simulink model "pokus07_video"  (R2023a)
settings: Solver=VariableStepAuto  StartTime=0.0  StopTime=10.0  RelTol=1e-3
undefined symbols (not defined in the file): c
libraries: Miscellaneous x840, Memory_Blocks_Lib x251, Decoders_Lib x10, simulink_extras x10, Counters_Lib x4, Bit_Multiplexers_Lib x1, Byte_Multiplexers_Lib x1
(part 3 of 5)

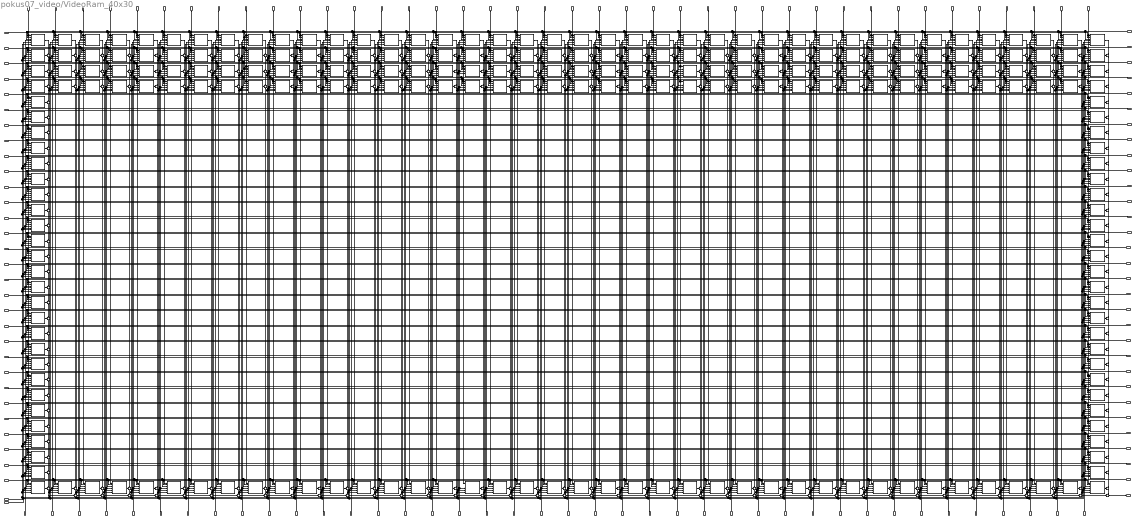
== system pokus07_video/VideoRam_40x30 ==
  RR29 : Inport
  RR28 : Inport  Port=2
  RR27 : Inport  Port=3
  RR26 : Inport  Port=4
  RR25 : Inport  Port=5
  RR24 : Inport  Port=6
  RR23 : Inport  Port=7
  RR22 : Inport  Port=8
  RR21 : Inport  Port=9
  RR20 : Inport  Port=10
  RR19 : Inport  Port=11
  RR18 : Inport  Port=12
  RR17 : Inport  Port=13
  RR16 : Inport  Port=14
  RR15 : Inport  Port=15
  RR14 : Inport  Port=16
  RR13 : Inport  Port=17
  RR12 : Inport  Port=18
  RR11 : Inport  Port=19
  RR10 : Inport  Port=20
  RR09 : Inport  Port=21
  RR08 : Inport  Port=22
  RR07 : Inport  Port=23
  RR06 : Inport  Port=24
  RR05 : Inport  Port=25
  RR04 : Inport  Port=26
  RR03 : Inport  Port=27
  RR02 : Inport  Port=28
  RR01 : Inport  Port=29
  RR00 : Inport  Port=30
  OrdNumIn(2B) : Inport  Port=31
  CLK : Inport  Port=32
  RC39 : Inport  Port=33
  RC38 : Inport  Port=34
  RC37 : Inport  Port=35
  RC36 : Inport  Port=36
  RC35 : Inport  Port=37
  RC34 : Inport  Port=38
  RC33 : Inport  Port=39
  RC32 : Inport  Port=40
  RC31 : Inport  Port=41
  RC30 : Inport  Port=42
  RC29 : Inport  Port=43
  RC28 : Inport  Port=44
  RC27 : Inport  Port=45
  RC26 : Inport  Port=46
  RC25 : Inport  Port=47
  RC24 : Inport  Port=48
  RC23 : Inport  Port=49
  RC22 : Inport  Port=50
  RC21 : Inport  Port=51
  RC20 : Inport  Port=52
  RC19 : Inport  Port=53
  RC18 : Inport  Port=54
  RC17 : Inport  Port=55
  RC16 : Inport  Port=56
  RC15 : Inport  Port=57
  RC14 : Inport  Port=58
  RC13 : Inport  Port=59
  RC12 : Inport  Port=60
  RC11 : Inport  Port=61
  RC10 : Inport  Port=62
  RC09 : Inport  Port=63
  RC08 : Inport  Port=64
  RC07 : Inport  Port=65
  RC06 : Inport  Port=66
  RC05 : Inport  Port=67
  RC04 : Inport  Port=68
  RC03 : Inport  Port=69
  RC02 : Inport  Port=70
  RC01 : Inport  Port=71
  RC00 : Inport  Port=72
  WC39 : Inport  Port=73
  WC38 : Inport  Port=74
  WC37 : Inport  Port=75
  WC36 : Inport  Port=76
  WC35 : Inport  Port=77
  WC34 : Inport  Port=78
  WC33 : Inport  Port=79
  WC32 : Inport  Port=80
  WC31 : Inport  Port=81
  WC30 : Inport  Port=82
  WC29 : Inport  Port=83
  WC28 : Inport  Port=84
  WC27 : Inport  Port=85
  WC26 : Inport  Port=86
  WC25 : Inport  Port=87
  WC24 : Inport  Port=88
  WC23 : Inport  Port=89
  WC22 : Inport  Port=90
  WC21 : Inport  Port=91
  WC20 : Inport  Port=92
  WC19 : Inport  Port=93
  WC18 : Inport  Port=94
  WC17 : Inport  Port=95
  WC16 : Inport  Port=96
  WC15 : Inport  Port=97
  WC14 : Inport  Port=98
  WC13 : Inport  Port=99
  WC12 : Inport  Port=100
  WC11 : Inport  Port=101
  WC10 : Inport  Port=102
  WC09 : Inport  Port=103
  WC08 : Inport  Port=104
  WC07 : Inport  Port=105
  WC06 : Inport  Port=106
  WC05 : Inport  Port=107
  WC04 : Inport  Port=108
  WC03 : Inport  Port=109
  WC02 : Inport  Port=110
  WC01 : Inport  Port=111
  WC00 : Inport  Port=112
  WR29 : Inport  Port=113
  WR28 : Inport  Port=114
  WR27 : Inport  Port=115
  WR26 : Inport  Port=116
  WR25 : Inport  Port=117
  WR24 : Inport  Port=118
  WR23 : Inport  Port=119
  WR22 : Inport  Port=120
  WR21 : Inport  Port=121
  WR20 : Inport  Port=122
  WR19 : Inport  Port=123
  WR18 : Inport  Port=124
  WR17 : Inport  Port=125
  WR16 : Inport  Port=126
  WR15 : Inport  Port=127
  WR14 : Inport  Port=128
  WR13 : Inport  Port=129
  WR12 : Inport  Port=130
  WR11 : Inport  Port=131
  WR10 : Inport  Port=132
  WR09 : Inport  Port=133
  WR08 : Inport  Port=134
  WR07 : Inport  Port=135
  WR06 : Inport  Port=136
  WR05 : Inport  Port=137
  WR04 : Inport  Port=138
  WR03 : Inport  Port=139
  WR02 : Inport  Port=140
  WR01 : Inport  Port=141
  WR00 : Inport  Port=142
  Byte_TwoBusAccess{,1..249} (250 alike) : Memory_Blocks_Lib/Byte_TwoBusAccess  SystemSampleTime=-1  VariantActivationTime=update diagram  Latency=0  AutoFrameSizeCalculation=off
  Merge2_Simulated{1..15,17..64,66..67,74..75,88..89,92..93,100,102,105..107,112..114,116..117,123..124,126..127,129..131,133..137,140..146,151,154..155,158..161,163..164,167..174,179,184,189,191..193,195..201,203..205,207..209,211..213,215,217..219,222..225,227..233,235..237,239..241,243..245,247,249..251,254..257,259..265,267..269,271..273,275..277,279,281..283,286..289,291..297,299..301,303..305,307..309,311..348} (249 alike) : Miscellaneous/Merge2_Simulated  SystemSampleTime=-1  VariantActivationTime=update diagram  Latency=0  AutoFrameSizeCalculation=off
      settings: PortSchema="{\"entries\":[{\"content\":{\"sides\":[{\"content\":{\"connectorIds\":[\"In1\"]},\"type\":\"ConnectorPlacement.EquallySpacedRectSide\",\"uuid\":\"74758995-5ec8-49f8-a534-c3a678c5c312\"},{\"content\":{\"side\":\"RIGHT\"},\"type\":\"ConnectorPlacement.EquallySpacedRectSide\",\"uuid\":\"c467dbeb-9f00-48b9-a78d-a08162163a10\"},{\"content\":{\"connectorIds\":[\"Out1\"],\"side\":\"TOP\"},\"type\":\"ConnectorPlacement.EquallySpacedRectSide\",\"uuid\":\"39dea3b5-6733-4ade-ab22-e62d310be187\"},{\"content\":{\"connectorIds\":[\"In2\"],\"side\":\"BOTTOM\"},\"type\":\"ConnectorPlacement.EquallySpacedRectSide\",\"uuid\":\"73149fc1-24d9-4bdc-92e2-12fb1d742836\"}]},\"type\":\"ConnectorPlacement.EquallySpacedConnector\",\"uuid\":\"fd2226dc-a4d3-43ad-9cda-54babd09ac78\"}],\"packageUris\":[\"http://schema.mathworks.com/mf0/Connector/R2020b\"],\"version\":\"1.0\"}"
  OrdNumOut(1B) : Outport
  wires:
  Byte_TwoBusAccess52/1 -> Merge2_Simulated1/1
  Byte_TwoBusAccess132/1 -> Merge2_Simulated3/1
  Byte_TwoBusAccess92/1 -> Merge2_Simulated2/1
  Merge2_Simulated2/1 -> Merge2_Simulated3/2
  Merge2_Simulated1/1 -> Merge2_Simulated2/2
  Byte_TwoBusAccess2/1 -> Merge2_Simulated1/2
  Byte_TwoBusAccess121/1 -> Merge2_Simulated7/1
  Merge2_Simulated5/1 -> Merge2_Simulated6/2
  Byte_TwoBusAccess1/1 -> Merge2_Simulated5/2
  Byte_TwoBusAccess81/1 -> Merge2_Simulated6/1
  Byte_TwoBusAccess41/1 -> Merge2_Simulated5/1
  Merge2_Simulated6/1 -> Merge2_Simulated7/2
  Byte_TwoBusAccess120/1 -> Merge2_Simulated11/1
  Merge2_Simulated9/1 -> Merge2_Simulated10/2
  Byte_TwoBusAccess/1 -> Merge2_Simulated9/2
  Byte_TwoBusAccess80/1 -> Merge2_Simulated10/1
  Byte_TwoBusAccess40/1 -> Merge2_Simulated9/1
  Merge2_Simulated10/1 -> Merge2_Simulated11/2
  Byte_TwoBusAccess143/1 -> Merge2_Simulated15/1
  Merge2_Simulated13/1 -> Merge2_Simulated14/2
  Byte_TwoBusAccess3/1 -> Merge2_Simulated13/2
  Byte_TwoBusAccess103/1 -> Merge2_Simulated14/1
  Byte_TwoBusAccess63/1 -> Merge2_Simulated13/1
  Merge2_Simulated14/1 -> Merge2_Simulated15/2
  Merge2_Simulated18/1 -> Merge2_Simulated19/2
  Merge2_Simulated30/1 -> Merge2_Simulated31/2
  Merge2_Simulated31/1 -> Merge2_Simulated18/2
  Byte_TwoBusAccess228/1 -> Merge2_Simulated19/1
  Byte_TwoBusAccess225/1 -> Merge2_Simulated30/1
  Byte_TwoBusAccess227/1 -> Merge2_Simulated18/1
  Byte_TwoBusAccess226/1 -> Merge2_Simulated31/1
  RC01/1 -> Byte_TwoBusAccess1/1, Byte_TwoBusAccess41/1, Byte_TwoBusAccess81/1, Byte_TwoBusAccess161/1, Byte_TwoBusAccess121/1
  Merge2_Simulated11/1 -> Merge2_Simulated30/2
  Merge2_Simulated34/1 -> Merge2_Simulated35/2
  Merge2_Simulated62/1 -> Merge2_Simulated63/2
  Merge2_Simulated63/1 -> Merge2_Simulated34/2
  Byte_TwoBusAccess235/1 -> Merge2_Simulated42/1
  Byte_TwoBusAccess236/1 -> Merge2_Simulated43/1
  Byte_TwoBusAccess234/1 -> Merge2_Simulated57/1
  Merge2_Simulated56/1 -> Merge2_Simulated57/2
  Byte_TwoBusAccess229/1 -> Merge2_Simulated62/1
  Byte_TwoBusAccess231/1 -> Merge2_Simulated34/1
  Byte_TwoBusAccess230/1 -> Merge2_Simulated63/1
  Byte_TwoBusAccess232/1 -> Merge2_Simulated35/1
  Merge2_Simulated35/1 -> Merge2_Simulated56/2
  Merge2_Simulated57/1 -> Merge2_Simulated42/2
  Merge2_Simulated42/1 -> Merge2_Simulated43/2
  Byte_TwoBusAccess233/1 -> Merge2_Simulated56/1
  Merge2_Simulated19/1 -> Merge2_Simulated62/2
  Merge2_Simulated66/1 -> Merge2_Simulated67/2
  Merge2_Simulated126/1 -> Merge2_Simulated127/2
  Merge2_Simulated127/1 -> Merge2_Simulated66/2
  Merge2_Simulated75/1 -> Merge2_Simulated123/2
  Byte_TwoBusAccess249/1 -> Merge2_Simulated116/1
  Merge2_Simulated93/1 -> Merge2_Simulated116/2
  Byte_TwoBusAccess160/1 -> Merge2_Simulated117/1
  Byte_TwoBusAccess183/1 -> Merge2_Simulated105/1
  Merge2_Simulated124/1 -> Merge2_Simulated92/2
  Merge2_Simulated123/1 -> Merge2_Simulated124/2
  Merge2_Simulated92/1 -> Merge2_Simulated93/2
  Byte_TwoBusAccess245/1 -> Merge2_Simulated123/1
  Merge2_Simulated15/1 -> Merge2_Simulated105/2
  Merge2_Simulated116/1 -> Merge2_Simulated117/2
  WC01/1 -> Byte_TwoBusAccess161/4, Byte_TwoBusAccess121/4, Byte_TwoBusAccess81/4, Byte_TwoBusAccess41/4, Byte_TwoBusAccess1/4
  WC00/1 -> Byte_TwoBusAccess160/4, Byte_TwoBusAccess249/4, Byte_TwoBusAccess248/4, Byte_TwoBusAccess247/4, Byte_TwoBusAccess246/4, Byte_TwoBusAccess245/4, Byte_TwoBusAccess244/4, Byte_TwoBusAccess243/4, Byte_TwoBusAccess242/4, Byte_TwoBusAccess241/4, Byte_TwoBusAccess240/4, Byte_TwoBusAccess239/4, Byte_TwoBusAccess238/4, Byte_TwoBusAccess237/4, Byte_TwoBusAccess236/4, Byte_TwoBusAccess235/4, Byte_TwoBusAccess234/4, Byte_TwoBusAccess233/4, Byte_TwoBusAccess232/4, Byte_TwoBusAccess231/4, Byte_TwoBusAccess230/4, Byte_TwoBusAccess229/4, Byte_TwoBusAccess228/4, Byte_TwoBusAccess227/4, Byte_TwoBusAccess226/4, Byte_TwoBusAccess225/4, Byte_TwoBusAccess120/4, Byte_TwoBusAccess80/4, Byte_TwoBusAccess40/4, Byte_TwoBusAccess/4
  Merge2_Simulated7/1 -> Merge2_Simulated112/2
  Byte_TwoBusAccess172/1 -> Merge2_Simulated100/1
  Merge2_Simulated3/1 -> Merge2_Simulated100/2
  Byte_TwoBusAccess243/1 -> Merge2_Simulated74/1
  Byte_TwoBusAccess244/1 -> Merge2_Simulated75/1
  Byte_TwoBusAccess242/1 -> Merge2_Simulated89/1
  Merge2_Simulated88/1 -> Merge2_Simulated89/2
  Byte_TwoBusAccess237/1 -> Merge2_Simulated126/1
  Byte_TwoBusAccess239/1 -> Merge2_Simulated66/1
  Byte_TwoBusAccess238/1 -> Merge2_Simulated127/1
  Byte_TwoBusAccess161/1 -> Merge2_Simulated112/1
  Byte_TwoBusAccess240/1 -> Merge2_Simulated67/1
  Merge2_Simulated67/1 -> Merge2_Simulated88/2
  Merge2_Simulated89/1 -> Merge2_Simulated74/2
  Byte_TwoBusAccess241/1 -> Merge2_Simulated88/1
  Merge2_Simulated74/1 -> Merge2_Simulated75/2
  Byte_TwoBusAccess246/1 -> Merge2_Simulated124/1
  RC02/1 -> Byte_TwoBusAccess2/1, Byte_TwoBusAccess52/1, Byte_TwoBusAccess92/1, Byte_TwoBusAccess172/1, Byte_TwoBusAccess132/1
  Byte_TwoBusAccess247/1 -> Merge2_Simulated92/1
  RC00/1 -> Byte_TwoBusAccess/1, Byte_TwoBusAccess40/1, Byte_TwoBusAccess80/1, Byte_TwoBusAccess120/1, Byte_TwoBusAccess225/1, Byte_TwoBusAccess226/1, Byte_TwoBusAccess227/1, Byte_TwoBusAccess228/1, Byte_TwoBusAccess229/1, Byte_TwoBusAccess230/1, Byte_TwoBusAccess231/1, Byte_TwoBusAccess232/1, Byte_TwoBusAccess233/1, Byte_TwoBusAccess234/1, Byte_TwoBusAccess235/1, Byte_TwoBusAccess236/1, Byte_TwoBusAccess237/1, Byte_TwoBusAccess238/1, Byte_TwoBusAccess239/1, Byte_TwoBusAccess240/1, Byte_TwoBusAccess241/1, Byte_TwoBusAccess242/1, Byte_TwoBusAccess243/1, Byte_TwoBusAccess244/1, Byte_TwoBusAccess245/1, Byte_TwoBusAccess246/1, Byte_TwoBusAccess247/1, Byte_TwoBusAccess248/1, Byte_TwoBusAccess249/1, Byte_TwoBusAccess160/1
  Byte_TwoBusAccess248/1 -> Merge2_Simulated93/1
  Merge2_Simulated43/1 -> Merge2_Simulated126/2
  Merge2_Simulated129/1 -> Merge2_Simulated140/2
  Byte_TwoBusAccess156/1 -> Merge2_Simulated151/1
  Merge2_Simulated133/1 -> Merge2_Simulated134/2
  Merge2_Simulated130/1 -> Merge2_Simulated131/2
  Byte_TwoBusAccess4/1 -> Merge2_Simulated191/2
  Merge2_Simulated191/1 -> Merge2_Simulated130/2
  Merge2_Simulated134/1 -> Merge2_Simulated135/2
  Merge2_Simulated184/1 -> Merge2_Simulated189/2
  Merge2_Simulated173/1 -> Merge2_Simulated184/2
  Byte_TwoBusAccess117/1 -> Merge2_Simulated134/1
  Byte_TwoBusAccess76/1 -> Merge2_Simulated129/1
  Byte_TwoBusAccess5/1 -> Merge2_Simulated173/2
  Byte_TwoBusAccess157/1 -> Merge2_Simulated135/1
  Byte_TwoBusAccess7/1 -> Merge2_Simulated133/2
  Byte_TwoBusAccess114/1 -> Merge2_Simulated130/1
  Byte_TwoBusAccess74/1 -> Merge2_Simulated191/1
  Byte_TwoBusAccess154/1 -> Merge2_Simulated131/1
  Byte_TwoBusAccess115/1 -> Merge2_Simulated184/1
  Byte_TwoBusAccess155/1 -> Merge2_Simulated189/1
  Byte_TwoBusAccess116/1 -> Merge2_Simulated140/1
  RC06/1 -> Byte_TwoBusAccess6/1, Byte_TwoBusAccess76/1, Byte_TwoBusAccess116/1, Byte_TwoBusAccess196/1, Byte_TwoBusAccess156/1
  Byte_TwoBusAccess75/1 -> Merge2_Simulated173/1
  Byte_TwoBusAccess6/1 -> Merge2_Simulated129/2
  RC04/1 -> Byte_TwoBusAccess4/1, Byte_TwoBusAccess74/1, Byte_TwoBusAccess114/1, Byte_TwoBusAccess194/1, Byte_TwoBusAccess154/1
  Byte_TwoBusAccess77/1 -> Merge2_Simulated133/1
  Merge2_Simulated140/1 -> Merge2_Simulated151/2
  WC13/1 -> Byte_TwoBusAccess165/4, Byte_TwoBusAccess125/4, Byte_TwoBusAccess85/4, Byte_TwoBusAccess45/4, Byte_TwoBusAccess13/4
  WC14/1 -> Byte_TwoBusAccess166/4, Byte_TwoBusAccess126/4, Byte_TwoBusAccess86/4, Byte_TwoBusAccess46/4, Byte_TwoBusAccess14/4
  WC15/1 -> Byte_TwoBusAccess167/4, Byte_TwoBusAccess127/4, Byte_TwoBusAccess87/4, Byte_TwoBusAccess47/4, Byte_TwoBusAccess15/4
  Byte_TwoBusAccess14/1 -> Merge2_Simulated113/2
  WC12/1 -> Byte_TwoBusAccess164/4, Byte_TwoBusAccess124/4, Byte_TwoBusAccess84/4, Byte_TwoBusAccess44/4, Byte_TwoBusAccess12/4
  Merge2_Simulated208/1 -> Merge2_Simulated209/2
  Byte_TwoBusAccess47/1 -> Merge2_Simulated195/1
  Byte_TwoBusAccess45/1 -> Merge2_Simulated203/1
  Byte_TwoBusAccess8/1 -> Merge2_Simulated215/2
  Merge2_Simulated207/1 -> Merge2_Simulated192/2
  Byte_TwoBusAccess12/1 -> Merge2_Simulated207/2
  Byte_TwoBusAccess119/1 -> Merge2_Simulated212/1
  Merge2_Simulated195/1 -> Merge2_Simulated196/2
  Byte_TwoBusAccess126/1 -> Merge2_Simulated201/1
  WC11/1 -> Byte_TwoBusAccess163/4, Byte_TwoBusAccess123/4, Byte_TwoBusAccess83/4, Byte_TwoBusAccess43/4, Byte_TwoBusAccess11/4
  Merge2_Simulated102/1 -> Merge2_Simulated208/2
  Byte_TwoBusAccess10/1 -> Merge2_Simulated102/2
  Byte_TwoBusAccess123/1 -> Merge2_Simulated200/1
  Merge2_Simulated212/1 -> Merge2_Simulated213/2
  Byte_TwoBusAccess122/1 -> Merge2_Simulated209/1
  Byte_TwoBusAccess127/1 -> Merge2_Simulated197/1
  Byte_TwoBusAccess46/1 -> Merge2_Simulated113/1
  Merge2_Simulated204/1 -> Merge2_Simulated205/2
  RC12/1 -> Byte_TwoBusAccess12/1, Byte_TwoBusAccess44/1, Byte_TwoBusAccess84/1, Byte_TwoBusAccess164/1, Byte_TwoBusAccess124/1
  Byte_TwoBusAccess43/1 -> Merge2_Simulated114/1
  Merge2_Simulated113/1 -> Merge2_Simulated199/2
  WC09/1 -> Byte_TwoBusAccess199/4, Byte_TwoBusAccess159/4, Byte_TwoBusAccess119/4, Byte_TwoBusAccess79/4, Byte_TwoBusAccess9/4
  Byte_TwoBusAccess159/1 -> Merge2_Simulated213/1
  Merge2_Simulated192/1 -> Merge2_Simulated193/2
  Merge2_Simulated114/1 -> Merge2_Simulated198/2
  Byte_TwoBusAccess84/1 -> Merge2_Simulated192/1
  RC13/1 -> Byte_TwoBusAccess13/1, Byte_TwoBusAccess45/1, Byte_TwoBusAccess85/1, Byte_TwoBusAccess165/1, Byte_TwoBusAccess125/1
  Byte_TwoBusAccess87/1 -> Merge2_Simulated196/1
  WC10/1 -> Byte_TwoBusAccess162/4, Byte_TwoBusAccess122/4, Byte_TwoBusAccess82/4, Byte_TwoBusAccess42/4, Byte_TwoBusAccess10/4
  Byte_TwoBusAccess85/1 -> Merge2_Simulated204/1
  Merge2_Simulated196/1 -> Merge2_Simulated197/2
  RC15/1 -> Byte_TwoBusAccess15/1, Byte_TwoBusAccess47/1, Byte_TwoBusAccess87/1, Byte_TwoBusAccess167/1, Byte_TwoBusAccess127/1
  Merge2_Simulated199/1 -> Merge2_Simulated201/2
  RC14/1 -> Byte_TwoBusAccess14/1, Byte_TwoBusAccess46/1, Byte_TwoBusAccess86/1, Byte_TwoBusAccess166/1, Byte_TwoBusAccess126/1
  Merge2_Simulated203/1 -> Merge2_Simulated204/2
  WR02/1 -> Byte_TwoBusAccess113/3, Byte_TwoBusAccess112/3, Byte_TwoBusAccess111/3, Byte_TwoBusAccess110/3, Byte_TwoBusAccess109/3, Byte_TwoBusAccess108/3, Byte_TwoBusAccess98/3, Byte_TwoBusAccess97/3, Byte_TwoBusAccess96/3, Byte_TwoBusAccess95/3, Byte_TwoBusAccess94/3, Byte_TwoBusAccess93/3, Byte_TwoBusAccess91/3, Byte_TwoBusAccess90/3, Byte_TwoBusAccess107/3, Byte_TwoBusAccess106/3, Byte_TwoBusAccess105/3, Byte_TwoBusAccess104/3, Byte_TwoBusAccess102/3, Byte_TwoBusAccess101/3, Byte_TwoBusAccess100/3, Byte_TwoBusAccess99/3, Byte_TwoBusAccess89/3, Byte_TwoBusAccess88/3, Byte_TwoBusAccess87/3, Byte_TwoBusAccess86/3, Byte_TwoBusAccess85/3, Byte_TwoBusAccess84/3, Byte_TwoBusAccess83/3, Byte_TwoBusAccess82/3, Byte_TwoBusAccess119/3, Byte_TwoBusAccess118/3, Byte_TwoBusAccess117/3, Byte_TwoBusAccess116/3, Byte_TwoBusAccess115/3, Byte_TwoBusAccess114/3, Byte_TwoBusAccess103/3, Byte_TwoBusAccess92/3, Byte_TwoBusAccess81/3, Byte_TwoBusAccess80/3
  RC10/1 -> Byte_TwoBusAccess10/1, Byte_TwoBusAccess42/1, Byte_TwoBusAccess82/1, Byte_TwoBusAccess162/1, Byte_TwoBusAccess122/1
  Byte_TwoBusAccess118/1 -> Merge2_Simulated106/1
  WR03/1 -> Byte_TwoBusAccess153/3, Byte_TwoBusAccess152/3, Byte_TwoBusAccess151/3, Byte_TwoBusAccess150/3, Byte_TwoBusAccess149/3, Byte_TwoBusAccess148/3, Byte_TwoBusAccess138/3, Byte_TwoBusAccess137/3, Byte_TwoBusAccess136/3, Byte_TwoBusAccess135/3, Byte_TwoBusAccess134/3, Byte_TwoBusAccess133/3, Byte_TwoBusAccess131/3, Byte_TwoBusAccess130/3, Byte_TwoBusAccess147/3, Byte_TwoBusAccess146/3, Byte_TwoBusAccess145/3, Byte_TwoBusAccess144/3, Byte_TwoBusAccess142/3, Byte_TwoBusAccess141/3, Byte_TwoBusAccess140/3, Byte_TwoBusAccess139/3, Byte_TwoBusAccess129/3, Byte_TwoBusAccess128/3, Byte_TwoBusAccess127/3, Byte_TwoBusAccess126/3, Byte_TwoBusAccess125/3, Byte_TwoBusAccess124/3, Byte_TwoBusAccess123/3, Byte_TwoBusAccess122/3, Byte_TwoBusAccess159/3, Byte_TwoBusAccess158/3, Byte_TwoBusAccess157/3, Byte_TwoBusAccess156/3, Byte_TwoBusAccess155/3, Byte_TwoBusAccess154/3, Byte_TwoBusAccess143/3, Byte_TwoBusAccess132/3, Byte_TwoBusAccess121/3, Byte_TwoBusAccess120/3
  RC09/1 -> Byte_TwoBusAccess9/1, Byte_TwoBusAccess79/1, Byte_TwoBusAccess119/1, Byte_TwoBusAccess199/1, Byte_TwoBusAccess159/1
  RC11/1 -> Byte_TwoBusAccess11/1, Byte_TwoBusAccess43/1, Byte_TwoBusAccess83/1, Byte_TwoBusAccess163/1, Byte_TwoBusAccess123/1
  Byte_TwoBusAccess11/1 -> Merge2_Simulated114/2
  Byte_TwoBusAccess124/1 -> Merge2_Simulated193/1
  Byte_TwoBusAccess82/1 -> Merge2_Simulated208/1
  Merge2_Simulated106/1 -> Merge2_Simulated107/2
  Byte_TwoBusAccess44/1 -> Merge2_Simulated207/1
  Byte_TwoBusAccess15/1 -> Merge2_Simulated195/2
  Byte_TwoBusAccess86/1 -> Merge2_Simulated199/1
  Byte_TwoBusAccess9/1 -> Merge2_Simulated211/2
  Merge2_Simulated198/1 -> Merge2_Simulated200/2
  Byte_TwoBusAccess42/1 -> Merge2_Simulated102/1
  Byte_TwoBusAccess78/1 -> Merge2_Simulated215/1
  Byte_TwoBusAccess83/1 -> Merge2_Simulated198/1
  Byte_TwoBusAccess13/1 -> Merge2_Simulated203/2
  Byte_TwoBusAccess158/1 -> Merge2_Simulated107/1
  Merge2_Simulated211/1 -> Merge2_Simulated212/2
  Byte_TwoBusAccess125/1 -> Merge2_Simulated205/1
  Byte_TwoBusAccess79/1 -> Merge2_Simulated211/1
  Merge2_Simulated215/1 -> Merge2_Simulated106/2
  WC21/1 -> Byte_TwoBusAccess182/4, Byte_TwoBusAccess142/4, Byte_TwoBusAccess102/4, Byte_TwoBusAccess62/4, Byte_TwoBusAccess29/4
  WC22/1 -> Byte_TwoBusAccess184/4, Byte_TwoBusAccess144/4, Byte_TwoBusAccess104/4, Byte_TwoBusAccess64/4, Byte_TwoBusAccess30/4
  WC23/1 -> Byte_TwoBusAccess185/4, Byte_TwoBusAccess145/4, Byte_TwoBusAccess105/4, Byte_TwoBusAccess65/4, Byte_TwoBusAccess31/4
  Byte_TwoBusAccess30/1 -> Merge2_Simulated222/2
  WC20/1 -> Byte_TwoBusAccess181/4, Byte_TwoBusAccess141/4, Byte_TwoBusAccess101/4, Byte_TwoBusAccess61/4, Byte_TwoBusAccess28/4
  Merge2_Simulated240/1 -> Merge2_Simulated241/2
  Byte_TwoBusAccess65/1 -> Merge2_Simulated227/1
  Byte_TwoBusAccess62/1 -> Merge2_Simulated235/1
  Byte_TwoBusAccess16/1 -> Merge2_Simulated247/2
  Merge2_Simulated239/1 -> Merge2_Simulated224/2
  Byte_TwoBusAccess28/1 -> Merge2_Simulated239/2
  Byte_TwoBusAccess89/1 -> Merge2_Simulated244/1
  Merge2_Simulated227/1 -> Merge2_Simulated228/2
  Byte_TwoBusAccess144/1 -> Merge2_Simulated233/1
  WC19/1 -> Byte_TwoBusAccess180/4, Byte_TwoBusAccess140/4, Byte_TwoBusAccess100/4, Byte_TwoBusAccess60/4, Byte_TwoBusAccess27/4
  Merge2_Simulated217/1 -> Merge2_Simulated240/2
  Byte_TwoBusAccess26/1 -> Merge2_Simulated217/2
  Byte_TwoBusAccess140/1 -> Merge2_Simulated232/1
  Merge2_Simulated244/1 -> Merge2_Simulated245/2
  Byte_TwoBusAccess139/1 -> Merge2_Simulated241/1
  Byte_TwoBusAccess145/1 -> Merge2_Simulated229/1
  Byte_TwoBusAccess64/1 -> Merge2_Simulated222/1
  Merge2_Simulated236/1 -> Merge2_Simulated237/2
  RC20/1 -> Byte_TwoBusAccess28/1, Byte_TwoBusAccess61/1, Byte_TwoBusAccess101/1, Byte_TwoBusAccess181/1, Byte_TwoBusAccess141/1
  Byte_TwoBusAccess60/1 -> Merge2_Simulated223/1
  Merge2_Simulated222/1 -> Merge2_Simulated231/2
  WC17/1 -> Byte_TwoBusAccess169/4, Byte_TwoBusAccess129/4, Byte_TwoBusAccess89/4, Byte_TwoBusAccess49/4, Byte_TwoBusAccess17/4
  Byte_TwoBusAccess129/1 -> Merge2_Simulated245/1
  Merge2_Simulated224/1 -> Merge2_Simulated225/2
  Merge2_Simulated223/1 -> Merge2_Simulated230/2
  Byte_TwoBusAccess101/1 -> Merge2_Simulated224/1
  Byte_TwoBusAccess105/1 -> Merge2_Simulated228/1
  WC18/1 -> Byte_TwoBusAccess179/4, Byte_TwoBusAccess139/4, Byte_TwoBusAccess99/4, Byte_TwoBusAccess59/4, Byte_TwoBusAccess26/4
  Byte_TwoBusAccess102/1 -> Merge2_Simulated236/1
  Merge2_Simulated228/1 -> Merge2_Simulated229/2
  RC23/1 -> Byte_TwoBusAccess31/1, Byte_TwoBusAccess65/1, Byte_TwoBusAccess105/1, Byte_TwoBusAccess185/1, Byte_TwoBusAccess145/1
  Merge2_Simulated231/1 -> Merge2_Simulated233/2
  RC22/1 -> Byte_TwoBusAccess30/1, Byte_TwoBusAccess64/1, Byte_TwoBusAccess104/1, Byte_TwoBusAccess184/1, Byte_TwoBusAccess144/1
  Merge2_Simulated235/1 -> Merge2_Simulated236/2
  RC18/1 -> Byte_TwoBusAccess26/1, Byte_TwoBusAccess59/1, Byte_TwoBusAccess99/1, Byte_TwoBusAccess179/1, Byte_TwoBusAccess139/1
  Byte_TwoBusAccess88/1 -> Merge2_Simulated218/1
  RC17/1 -> Byte_TwoBusAccess17/1, Byte_TwoBusAccess49/1, Byte_TwoBusAccess89/1, Byte_TwoBusAccess169/1, Byte_TwoBusAccess129/1
  RC19/1 -> Byte_TwoBusAccess27/1, Byte_TwoBusAccess60/1, Byte_TwoBusAccess100/1, Byte_TwoBusAccess180/1, Byte_TwoBusAccess140/1
  Byte_TwoBusAccess27/1 -> Merge2_Simulated223/2
  Byte_TwoBusAccess141/1 -> Merge2_Simulated225/1
  Byte_TwoBusAccess99/1 -> Merge2_Simulated240/1
  Merge2_Simulated218/1 -> Merge2_Simulated219/2
  Byte_TwoBusAccess61/1 -> Merge2_Simulated239/1
  Byte_TwoBusAccess31/1 -> Merge2_Simulated227/2
  Byte_TwoBusAccess104/1 -> Merge2_Simulated231/1
  Byte_TwoBusAccess17/1 -> Merge2_Simulated243/2
  Merge2_Simulated230/1 -> Merge2_Simulated232/2
  Byte_TwoBusAccess59/1 -> Merge2_Simulated217/1
  Byte_TwoBusAccess48/1 -> Merge2_Simulated247/1
  Byte_TwoBusAccess100/1 -> Merge2_Simulated230/1
  Byte_TwoBusAccess29/1 -> Merge2_Simulated235/2
  Byte_TwoBusAccess128/1 -> Merge2_Simulated219/1
  Merge2_Simulated243/1 -> Merge2_Simulated244/2
  Byte_TwoBusAccess142/1 -> Merge2_Simulated237/1
  Byte_TwoBusAccess49/1 -> Merge2_Simulated243/1
  Merge2_Simulated247/1 -> Merge2_Simulated218/2
  Merge2_Simulated279/1 -> Merge2_Simulated250/2
  Byte_TwoBusAccess134/1 -> Merge2_Simulated269/1
  Byte_TwoBusAccess146/1 -> Merge2_Simulated251/1
  Byte_TwoBusAccess66/1 -> Merge2_Simulated279/1
  Byte_TwoBusAccess50/1 -> Merge2_Simulated249/1
  Merge2_Simulated262/1 -> Merge2_Simulated264/2
  Byte_TwoBusAccess90/1 -> Merge2_Simulated272/1
  Merge2_Simulated250/1 -> Merge2_Simulated251/2
  Merge2_Simulated311/1 -> Merge2_Simulated282/2
  Byte_TwoBusAccess57/1 -> Merge2_Simulated311/1
  Byte_TwoBusAccess109/1 -> Merge2_Simulated294/1
  Byte_TwoBusAccess151/1 -> Merge2_Simulated301/1
  Byte_TwoBusAccess137/1 -> Merge2_Simulated283/1
  Byte_TwoBusAccess58/1 -> Merge2_Simulated307/1
  Byte_TwoBusAccess37/1 -> Merge2_Simulated299/2
  Merge2_Simulated307/1 -> Merge2_Simulated308/2
  Merge2_Simulated294/1 -> Merge2_Simulated296/2
  Byte_TwoBusAccess25/1 -> Merge2_Simulated307/2
  Byte_TwoBusAccess39/1 -> Merge2_Simulated291/2
  Byte_TwoBusAccess70/1 -> Merge2_Simulated303/1
  Byte_TwoBusAccess112/1 -> Merge2_Simulated295/1
  Byte_TwoBusAccess68/1 -> Merge2_Simulated281/1
  Byte_TwoBusAccess108/1 -> Merge2_Simulated304/1
  RC35/1 -> Byte_TwoBusAccess35/1, Byte_TwoBusAccess69/1, Byte_TwoBusAccess109/1, Byte_TwoBusAccess189/1, Byte_TwoBusAccess149/1
  Byte_TwoBusAccess35/1 -> Merge2_Simulated287/2
  Merge2_Simulated300/1 -> Merge2_Simulated301/2
  Byte_TwoBusAccess153/1 -> Merge2_Simulated293/1
  Merge2_Simulated308/1 -> Merge2_Simulated309/2
  Byte_TwoBusAccess149/1 -> Merge2_Simulated296/1
  Merge2_Simulated281/1 -> Merge2_Simulated304/2
  Byte_TwoBusAccess152/1 -> Merge2_Simulated297/1
  Byte_TwoBusAccess98/1 -> Merge2_Simulated308/1
  Merge2_Simulated303/1 -> Merge2_Simulated288/2
  Byte_TwoBusAccess36/1 -> Merge2_Simulated303/2
  Byte_TwoBusAccess71/1 -> Merge2_Simulated299/1
  Byte_TwoBusAccess24/1 -> Merge2_Simulated311/2
  Merge2_Simulated304/1 -> Merge2_Simulated305/2
  Byte_TwoBusAccess34/1 -> Merge2_Simulated281/2
  Byte_TwoBusAccess38/1 -> Merge2_Simulated286/2
  WC36/1 -> Byte_TwoBusAccess190/4, Byte_TwoBusAccess150/4, Byte_TwoBusAccess110/4, Byte_TwoBusAccess70/4, Byte_TwoBusAccess36/4
  WC38/1 -> Byte_TwoBusAccess192/4, Byte_TwoBusAccess152/4, Byte_TwoBusAccess112/4, Byte_TwoBusAccess72/4, Byte_TwoBusAccess38/4
  Byte_TwoBusAccess72/1 -> Merge2_Simulated286/1
  WR00/1 -> Byte_TwoBusAccess39/3, Byte_TwoBusAccess38/3, Byte_TwoBusAccess37/3, Byte_TwoBusAccess36/3, Byte_TwoBusAccess35/3, Byte_TwoBusAccess34/3, Byte_TwoBusAccess25/3, Byte_TwoBusAccess24/3, Byte_TwoBusAccess23/3, Byte_TwoBusAccess22/3, Byte_TwoBusAccess21/3, Byte_TwoBusAccess20/3, Byte_TwoBusAccess19/3, Byte_TwoBusAccess18/3, Byte_TwoBusAccess33/3, Byte_TwoBusAccess32/3, Byte_TwoBusAccess31/3, Byte_TwoBusAccess30/3, Byte_TwoBusAccess29/3, Byte_TwoBusAccess28/3, Byte_TwoBusAccess27/3, Byte_TwoBusAccess26/3, Byte_TwoBusAccess17/3, Byte_TwoBusAccess16/3, Byte_TwoBusAccess15/3, Byte_TwoBusAccess14/3, Byte_TwoBusAccess13/3, Byte_TwoBusAccess12/3, Byte_TwoBusAccess11/3, Byte_TwoBusAccess10/3, Byte_TwoBusAccess9/3, Byte_TwoBusAccess8/3, Byte_TwoBusAccess7/3, Byte_TwoBusAccess6/3, Byte_TwoBusAccess5/3, Byte_TwoBusAccess4/3, Byte_TwoBusAccess3/3, Byte_TwoBusAccess2/3, Byte_TwoBusAccess1/3, Byte_TwoBusAccess/3
  Byte_TwoBusAccess138/1 -> Merge2_Simulated309/1
  WC33/1 -> Byte_TwoBusAccess178/4, Byte_TwoBusAccess138/4, Byte_TwoBusAccess98/4, Byte_TwoBusAccess58/4, Byte_TwoBusAccess25/4
  Merge2_Simulated286/1 -> Merge2_Simulated295/2
  RC36/1 -> Byte_TwoBusAccess36/1, Byte_TwoBusAccess70/1, Byte_TwoBusAccess110/1, Byte_TwoBusAccess190/1, Byte_TwoBusAccess150/1
  Merge2_Simulated291/1 -> Merge2_Simulated292/2
  WC37/1 -> Byte_TwoBusAccess191/4, Byte_TwoBusAccess151/4, Byte_TwoBusAccess111/4, Byte_TwoBusAccess71/4, Byte_TwoBusAccess37/4
  WC30/1 -> Byte_TwoBusAccess175/4, Byte_TwoBusAccess135/4, Byte_TwoBusAccess95/4, Byte_TwoBusAccess55/4, Byte_TwoBusAccess22/4
  Byte_TwoBusAccess96/1 -> Merge2_Simulated260/1
  RC26/1 -> Byte_TwoBusAccess18/1, Byte_TwoBusAccess50/1, Byte_TwoBusAccess90/1, Byte_TwoBusAccess170/1, Byte_TwoBusAccess130/1
  CLK/1 -> Byte_TwoBusAccess160/6, Byte_TwoBusAccess249/6, Byte_TwoBusAccess248/6, Byte_TwoBusAccess247/6, Byte_TwoBusAccess246/6, Byte_TwoBusAccess245/6, Byte_TwoBusAccess244/6, Byte_TwoBusAccess243/6, Byte_TwoBusAccess242/6, Byte_TwoBusAccess241/6, Byte_TwoBusAccess240/6, Byte_TwoBusAccess239/6, Byte_TwoBusAccess238/6, Byte_TwoBusAccess237/6, Byte_TwoBusAccess236/6, Byte_TwoBusAccess235/6, Byte_TwoBusAccess234/6, Byte_TwoBusAccess233/6, Byte_TwoBusAccess232/6, Byte_TwoBusAccess231/6, Byte_TwoBusAccess230/6, Byte_TwoBusAccess229/6, Byte_TwoBusAccess228/6, Byte_TwoBusAccess227/6, Byte_TwoBusAccess226/6, Byte_TwoBusAccess225/6, Byte_TwoBusAccess120/6, Byte_TwoBusAccess80/6, Byte_TwoBusAccess40/6, Byte_TwoBusAccess/6, Byte_TwoBusAccess193/6, Byte_TwoBusAccess224/6, Byte_TwoBusAccess223/6, Byte_TwoBusAccess222/6, Byte_TwoBusAccess221/6, Byte_TwoBusAccess220/6, Byte_TwoBusAccess219/6, Byte_TwoBusAccess218/6, Byte_TwoBusAccess217/6, Byte_TwoBusAccess216/6, Byte_TwoBusAccess215/6, Byte_TwoBusAccess214/6, Byte_TwoBusAccess213/6, Byte_TwoBusAccess212/6, Byte_TwoBusAccess211/6, Byte_TwoBusAccess210/6, Byte_TwoBusAccess209/6, Byte_TwoBusAccess208/6, Byte_TwoBusAccess207/6, Byte_TwoBusAccess206/6, Byte_TwoBusAccess205/6, Byte_TwoBusAccess204/6, Byte_TwoBusAccess203/6, Byte_TwoBusAccess202/6, Byte_TwoBusAccess201/6, Byte_TwoBusAccess200/6, Byte_TwoBusAccess153/6, Byte_TwoBusAccess113/6, Byte_TwoBusAccess73/6, Byte_TwoBusAccess39/6, Byte_TwoBusAccess192/6, Byte_TwoBusAccess152/6, Byte_TwoBusAccess112/6, Byte_TwoBusAccess72/6, Byte_TwoBusAccess38/6, Byte_TwoBusAccess191/6, Byte_TwoBusAccess151/6, Byte_TwoBusAccess111/6, Byte_TwoBusAccess71/6, Byte_TwoBusAccess37/6, Byte_TwoBusAccess190/6, Byte_TwoBusAccess150/6, Byte_TwoBusAccess110/6, Byte_TwoBusAccess70/6, Byte_TwoBusAccess36/6, Byte_TwoBusAccess189/6, Byte_TwoBusAccess149/6, Byte_TwoBusAccess109/6, Byte_TwoBusAccess69/6, Byte_TwoBusAccess35/6, Byte_TwoBusAccess188/6, Byte_TwoBusAccess148/6, Byte_TwoBusAccess108/6, Byte_TwoBusAccess68/6, Byte_TwoBusAccess34/6, Byte_TwoBusAccess178/6, Byte_TwoBusAccess138/6, Byte_TwoBusAccess98/6, Byte_TwoBusAccess58/6, Byte_TwoBusAccess25/6, Byte_TwoBusAccess177/6, Byte_TwoBusAccess137/6, Byte_TwoBusAccess97/6, Byte_TwoBusAccess57/6, Byte_TwoBusAccess24/6, Byte_TwoBusAccess176/6, Byte_TwoBusAccess136/6, Byte_TwoBusAccess96/6, Byte_TwoBusAccess56/6, Byte_TwoBusAccess23/6, Byte_TwoBusAccess175/6, Byte_TwoBusAccess135/6, Byte_TwoBusAccess95/6, Byte_TwoBusAccess55/6, Byte_TwoBusAccess22/6, Byte_TwoBusAccess174/6, Byte_TwoBusAccess134/6, Byte_TwoBusAccess94/6, Byte_TwoBusAccess54/6, Byte_TwoBusAccess21/6, Byte_TwoBusAccess173/6, Byte_TwoBusAccess133/6, Byte_TwoBusAccess93/6, Byte_TwoBusAccess53/6, Byte_TwoBusAccess20/6, Byte_TwoBusAccess171/6, Byte_TwoBusAccess131/6, Byte_TwoBusAccess91/6, Byte_TwoBusAccess51/6, Byte_TwoBusAccess19/6, Byte_TwoBusAccess170/6, Byte_TwoBusAccess130/6, Byte_TwoBusAccess90/6, Byte_TwoBusAccess50/6, Byte_TwoBusAccess18/6, Byte_TwoBusAccess187/6, Byte_TwoBusAccess147/6, Byte_TwoBusAccess107/6, Byte_TwoBusAccess67/6, Byte_TwoBusAccess33/6, Byte_TwoBusAccess186/6, Byte_TwoBusAccess146/6, Byte_TwoBusAccess106/6, Byte_TwoBusAccess66/6, Byte_TwoBusAccess32/6, Byte_TwoBusAccess185/6, Byte_TwoBusAccess145/6, Byte_TwoBusAccess105/6, Byte_TwoBusAccess65/6, Byte_TwoBusAccess31/6, Byte_TwoBusAccess184/6, Byte_TwoBusAccess144/6, Byte_TwoBusAccess104/6, Byte_TwoBusAccess64/6, Byte_TwoBusAccess30/6, Byte_TwoBusAccess182/6, Byte_TwoBusAccess142/6, Byte_TwoBusAccess102/6, Byte_TwoBusAccess62/6, Byte_TwoBusAccess29/6, Byte_TwoBusAccess181/6, Byte_TwoBusAccess141/6, Byte_TwoBusAccess101/6, Byte_TwoBusAccess61/6, Byte_TwoBusAccess28/6, Byte_TwoBusAccess180/6, Byte_TwoBusAccess140/6, Byte_TwoBusAccess100/6, Byte_TwoBusAccess60/6, Byte_TwoBusAccess27/6, Byte_TwoBusAccess179/6, Byte_TwoBusAccess139/6, Byte_TwoBusAccess99/6, Byte_TwoBusAccess59/6, Byte_TwoBusAccess26/6, Byte_TwoBusAccess169/6, Byte_TwoBusAccess129/6, Byte_TwoBusAccess89/6, Byte_TwoBusAccess49/6, Byte_TwoBusAccess17/6, Byte_TwoBusAccess168/6, Byte_TwoBusAccess128/6, Byte_TwoBusAccess48/6, Byte_TwoBusAccess16/6, Byte_TwoBusAccess167/6, Byte_TwoBusAccess127/6, Byte_TwoBusAccess87/6, Byte_TwoBusAccess47/6, Byte_TwoBusAccess15/6, Byte_TwoBusAccess166/6, Byte_TwoBusAccess126/6, Byte_TwoBusAccess86/6, Byte_TwoBusAccess46/6, Byte_TwoBusAccess14/6, Byte_TwoBusAccess165/6, Byte_TwoBusAccess125/6, Byte_TwoBusAccess85/6, Byte_TwoBusAccess45/6, Byte_TwoBusAccess13/6, Byte_TwoBusAccess164/6, Byte_TwoBusAccess124/6, Byte_TwoBusAccess84/6, Byte_TwoBusAccess44/6, Byte_TwoBusAccess12/6, Byte_TwoBusAccess163/6, Byte_TwoBusAccess123/6, Byte_TwoBusAccess83/6, Byte_TwoBusAccess43/6, Byte_TwoBusAccess11/6, Byte_TwoBusAccess162/6, Byte_TwoBusAccess122/6, Byte_TwoBusAccess82/6, Byte_TwoBusAccess42/6, Byte_TwoBusAccess10/6, Byte_TwoBusAccess199/6, Byte_TwoBusAccess159/6, Byte_TwoBusAccess119/6, Byte_TwoBusAccess79/6, Byte_TwoBusAccess9/6, Byte_TwoBusAccess198/6, Byte_TwoBusAccess158/6, Byte_TwoBusAccess118/6, Byte_TwoBusAccess78/6, Byte_TwoBusAccess8/6, Byte_TwoBusAccess197/6, Byte_TwoBusAccess157/6, Byte_TwoBusAccess117/6, Byte_TwoBusAccess77/6, Byte_TwoBusAccess7/6, Byte_TwoBusAccess196/6, Byte_TwoBusAccess156/6, Byte_TwoBusAccess116/6, Byte_TwoBusAccess76/6, Byte_TwoBusAccess6/6, Byte_TwoBusAccess195/6, Byte_TwoBusAccess155/6, Byte_TwoBusAccess115/6, Byte_TwoBusAccess75/6, Byte_TwoBusAccess5/6, Byte_TwoBusAccess194/6, Byte_TwoBusAccess154/6, Byte_TwoBusAccess114/6, Byte_TwoBusAccess74/6, Byte_TwoBusAccess4/6, Byte_TwoBusAccess183/6, Byte_TwoBusAccess143/6, Byte_TwoBusAccess103/6, Byte_TwoBusAccess63/6, Byte_TwoBusAccess3/6, Byte_TwoBusAccess172/6, Byte_TwoBusAccess132/6, Byte_TwoBusAccess92/6, Byte_TwoBusAccess52/6, Byte_TwoBusAccess2/6, Byte_TwoBusAccess161/6, Byte_TwoBusAccess121/6, Byte_TwoBusAccess81/6, Byte_TwoBusAccess41/6, Byte_TwoBusAccess1/6
  WC35/1 -> Byte_TwoBusAccess189/4, Byte_TwoBusAccess149/4, Byte_TwoBusAccess109/4, Byte_TwoBusAccess69/4, Byte_TwoBusAccess35/4
  Merge2_Simulated267/1 -> Merge2_Simulated268/2
  Byte_TwoBusAccess95/1 -> Merge2_Simulated263/1
  RC27/1 -> Byte_TwoBusAccess19/1, Byte_TwoBusAccess51/1, Byte_TwoBusAccess91/1, Byte_TwoBusAccess171/1, Byte_TwoBusAccess131/1
  Byte_TwoBusAccess33/1 -> Merge2_Simulated275/2
  Byte_TwoBusAccess21/1 -> Merge2_Simulated267/2
  Merge2_Simulated275/1 -> Merge2_Simulated276/2
  Byte_TwoBusAccess53/1 -> Merge2_Simulated271/1
  RC30/1 -> Byte_TwoBusAccess22/1, Byte_TwoBusAccess55/1, Byte_TwoBusAccess95/1, Byte_TwoBusAccess175/1, Byte_TwoBusAccess135/1
  Merge2_Simulated292/1 -> Merge2_Simulated293/2
  RR00/1 -> Byte_TwoBusAccess/2, Byte_TwoBusAccess1/2, Byte_TwoBusAccess2/2, Byte_TwoBusAccess3/2, Byte_TwoBusAccess4/2, Byte_TwoBusAccess5/2, Byte_TwoBusAccess6/2, Byte_TwoBusAccess7/2, Byte_TwoBusAccess9/2, Byte_TwoBusAccess10/2, Byte_TwoBusAccess11/2, Byte_TwoBusAccess12/2, Byte_TwoBusAccess13/2, Byte_TwoBusAccess14/2, Byte_TwoBusAccess15/2, Byte_TwoBusAccess16/2, Byte_TwoBusAccess17/2, Byte_TwoBusAccess26/2, Byte_TwoBusAccess27/2, Byte_TwoBusAccess28/2, Byte_TwoBusAccess29/2, Byte_TwoBusAccess30/2, Byte_TwoBusAccess31/2, Byte_TwoBusAccess32/2, Byte_TwoBusAccess33/2, Byte_TwoBusAccess18/2, Byte_TwoBusAccess19/2, Byte_TwoBusAccess20/2, Byte_TwoBusAccess21/2, Byte_TwoBusAccess22/2, Byte_TwoBusAccess23/2, Byte_TwoBusAccess24/2, Byte_TwoBusAccess25/2, Byte_TwoBusAccess34/2, Byte_TwoBusAccess35/2, Byte_TwoBusAccess36/2, Byte_TwoBusAccess37/2, Byte_TwoBusAccess39/2, Byte_TwoBusAccess38/2, Byte_TwoBusAccess8/2, Byte_TwoBusAccess158/2, Byte_TwoBusAccess118/2
  Byte_TwoBusAccess91/1 -> Merge2_Simulated262/1
  WC34/1 -> Byte_TwoBusAccess188/4, Byte_TwoBusAccess148/4, Byte_TwoBusAccess108/4, Byte_TwoBusAccess68/4, Byte_TwoBusAccess34/4
  RR01/1 -> Byte_TwoBusAccess40/2, Byte_TwoBusAccess41/2, Byte_TwoBusAccess52/2, Byte_TwoBusAccess63/2, Byte_TwoBusAccess74/2, Byte_TwoBusAccess75/2, Byte_TwoBusAccess76/2, Byte_TwoBusAccess77/2, Byte_TwoBusAccess78/2, Byte_TwoBusAccess79/2, Byte_TwoBusAccess42/2, Byte_TwoBusAccess43/2, Byte_TwoBusAccess44/2, Byte_TwoBusAccess45/2, Byte_TwoBusAccess46/2, Byte_TwoBusAccess47/2, Byte_TwoBusAccess48/2, Byte_TwoBusAccess49/2, Byte_TwoBusAccess59/2, Byte_TwoBusAccess60/2, Byte_TwoBusAccess61/2, Byte_TwoBusAccess62/2, Byte_TwoBusAccess64/2, Byte_TwoBusAccess65/2, Byte_TwoBusAccess66/2, Byte_TwoBusAccess67/2, Byte_TwoBusAccess50/2, Byte_TwoBusAccess51/2, Byte_TwoBusAccess53/2, Byte_TwoBusAccess54/2, Byte_TwoBusAccess55/2, Byte_TwoBusAccess56/2, Byte_TwoBusAccess57/2, Byte_TwoBusAccess58/2, Byte_TwoBusAccess68/2, Byte_TwoBusAccess69/2, Byte_TwoBusAccess70/2, Byte_TwoBusAccess71/2, Byte_TwoBusAccess73/2, Byte_TwoBusAccess72/2
  RC25/1 -> Byte_TwoBusAccess33/1, Byte_TwoBusAccess67/1, Byte_TwoBusAccess107/1, Byte_TwoBusAccess187/1, Byte_TwoBusAccess147/1
  RR02/1 -> Byte_TwoBusAccess80/2, Byte_TwoBusAccess81/2, Byte_TwoBusAccess92/2, Byte_TwoBusAccess103/2, Byte_TwoBusAccess114/2, Byte_TwoBusAccess115/2, Byte_TwoBusAccess116/2, Byte_TwoBusAccess117/2, Byte_TwoBusAccess119/2, Byte_TwoBusAccess82/2, Byte_TwoBusAccess83/2, Byte_TwoBusAccess84/2, Byte_TwoBusAccess85/2, Byte_TwoBusAccess86/2, Byte_TwoBusAccess87/2, Byte_TwoBusAccess88/2, Byte_TwoBusAccess89/2, Byte_TwoBusAccess99/2, Byte_TwoBusAccess100/2, Byte_TwoBusAccess101/2, Byte_TwoBusAccess102/2, Byte_TwoBusAccess104/2, Byte_TwoBusAccess105/2, Byte_TwoBusAccess107/2, Byte_TwoBusAccess90/2, Byte_TwoBusAccess91/2, Byte_TwoBusAccess93/2, Byte_TwoBusAccess94/2, Byte_TwoBusAccess95/2, Byte_TwoBusAccess96/2, Byte_TwoBusAccess97/2, Byte_TwoBusAccess98/2, Byte_TwoBusAccess108/2, Byte_TwoBusAccess109/2, Byte_TwoBusAccess110/2, Byte_TwoBusAccess111/2, Byte_TwoBusAccess113/2, Byte_TwoBusAccess112/2
  Byte_TwoBusAccess148/1 -> Merge2_Simulated305/1
  Byte_TwoBusAccess69/1 -> Merge2_Simulated287/1
  Byte_TwoBusAccess110/1 -> Merge2_Simulated288/1
  WC29/1 -> Byte_TwoBusAccess174/4, Byte_TwoBusAccess134/4, Byte_TwoBusAccess94/4, Byte_TwoBusAccess54/4, Byte_TwoBusAccess21/4
  Byte_TwoBusAccess150/1 -> Merge2_Simulated289/1
  RC38/1 -> Byte_TwoBusAccess38/1, Byte_TwoBusAccess72/1, Byte_TwoBusAccess112/1, Byte_TwoBusAccess192/1, Byte_TwoBusAccess152/1
  Byte_TwoBusAccess113/1 -> Merge2_Simulated292/1
  Merge2_Simulated299/1 -> Merge2_Simulated300/2
  Merge2_Simulated260/1 -> Merge2_Simulated261/2
  Byte_TwoBusAccess94/1 -> Merge2_Simulated268/1
  Byte_TwoBusAccess111/1 -> Merge2_Simulated300/1
  Byte_TwoBusAccess106/1 -> Merge2_Simulated250/1
  Byte_TwoBusAccess73/1 -> Merge2_Simulated291/1
  Merge2_Simulated268/1 -> Merge2_Simulated269/2
  Byte_TwoBusAccess55/1 -> Merge2_Simulated254/1
  RC29/1 -> Byte_TwoBusAccess21/1, Byte_TwoBusAccess54/1, Byte_TwoBusAccess94/1, Byte_TwoBusAccess174/1, Byte_TwoBusAccess134/1
  Byte_TwoBusAccess67/1 -> Merge2_Simulated275/1
  WR01/1 -> Byte_TwoBusAccess73/3, Byte_TwoBusAccess72/3, Byte_TwoBusAccess71/3, Byte_TwoBusAccess70/3, Byte_TwoBusAccess69/3, Byte_TwoBusAccess68/3, Byte_TwoBusAccess58/3, Byte_TwoBusAccess57/3, Byte_TwoBusAccess56/3, Byte_TwoBusAccess55/3, Byte_TwoBusAccess54/3, Byte_TwoBusAccess53/3, Byte_TwoBusAccess51/3, Byte_TwoBusAccess50/3, Byte_TwoBusAccess67/3, Byte_TwoBusAccess66/3, Byte_TwoBusAccess65/3, Byte_TwoBusAccess64/3, Byte_TwoBusAccess62/3, Byte_TwoBusAccess61/3, Byte_TwoBusAccess60/3, Byte_TwoBusAccess59/3, Byte_TwoBusAccess49/3, Byte_TwoBusAccess48/3, Byte_TwoBusAccess47/3, Byte_TwoBusAccess46/3, Byte_TwoBusAccess45/3, Byte_TwoBusAccess44/3, Byte_TwoBusAccess43/3, Byte_TwoBusAccess42/3, Byte_TwoBusAccess79/3, Byte_TwoBusAccess78/3, Byte_TwoBusAccess77/3, Byte_TwoBusAccess76/3, Byte_TwoBusAccess75/3, Byte_TwoBusAccess74/3, Byte_TwoBusAccess63/3, Byte_TwoBusAccess52/3, Byte_TwoBusAccess41/3, Byte_TwoBusAccess40/3
  RR03/1 -> Byte_TwoBusAccess120/2, Byte_TwoBusAccess121/2, Byte_TwoBusAccess132/2, Byte_TwoBusAccess143/2, Byte_TwoBusAccess154/2, Byte_TwoBusAccess155/2, Byte_TwoBusAccess156/2, Byte_TwoBusAccess157/2, Byte_TwoBusAccess159/2, Byte_TwoBusAccess122/2, Byte_TwoBusAccess123/2, Byte_TwoBusAccess124/2, Byte_TwoBusAccess125/2, Byte_TwoBusAccess126/2, Byte_TwoBusAccess127/2, Byte_TwoBusAccess128/2, Byte_TwoBusAccess129/2, Byte_TwoBusAccess139/2, Byte_TwoBusAccess140/2, Byte_TwoBusAccess141/2, Byte_TwoBusAccess142/2, Byte_TwoBusAccess144/2, Byte_TwoBusAccess145/2, Byte_TwoBusAccess147/2, Byte_TwoBusAccess130/2, Byte_TwoBusAccess131/2, Byte_TwoBusAccess133/2, Byte_TwoBusAccess134/2, Byte_TwoBusAccess135/2, Byte_TwoBusAccess136/2, Byte_TwoBusAccess137/2, Byte_TwoBusAccess138/2, Byte_TwoBusAccess148/2, Byte_TwoBusAccess149/2, Byte_TwoBusAccess150/2, Byte_TwoBusAccess151/2, Byte_TwoBusAccess152/2, Byte_TwoBusAccess153/2
  Merge2_Simulated255/1 -> Merge2_Simulated262/2
  Byte_TwoBusAccess147/1 -> Merge2_Simulated277/1
  Byte_TwoBusAccess51/1 -> Merge2_Simulated255/1
  WC25/1 -> Byte_TwoBusAccess187/4, Byte_TwoBusAccess147/4, Byte_TwoBusAccess107/4, Byte_TwoBusAccess67/4, Byte_TwoBusAccess33/4
  RC34/1 -> Byte_TwoBusAccess34/1, Byte_TwoBusAccess68/1, Byte_TwoBusAccess108/1, Byte_TwoBusAccess188/1, Byte_TwoBusAccess148/1
  Byte_TwoBusAccess23/1 -> Merge2_Simulated259/2
  Merge2_Simulated295/1 -> Merge2_Simulated297/2
  Merge2_Simulated256/1 -> Merge2_Simulated257/2
  Merge2_Simulated263/1 -> Merge2_Simulated265/2
  WC26/1 -> Byte_TwoBusAccess170/4, Byte_TwoBusAccess130/4, Byte_TwoBusAccess90/4, Byte_TwoBusAccess50/4, Byte_TwoBusAccess18/4
  Byte_TwoBusAccess93/1 -> Merge2_Simulated256/1
  Byte_TwoBusAccess97/1 -> Merge2_Simulated282/1
  Byte_TwoBusAccess56/1 -> Merge2_Simulated259/1
  Merge2_Simulated272/1 -> Merge2_Simulated273/2
  WC28/1 -> Byte_TwoBusAccess173/4, Byte_TwoBusAccess133/4, Byte_TwoBusAccess93/4, Byte_TwoBusAccess53/4, Byte_TwoBusAccess20/4
  Merge2_Simulated288/1 -> Merge2_Simulated289/2
  Merge2_Simulated287/1 -> Merge2_Simulated294/2
  Merge2_Simulated276/1 -> Merge2_Simulated277/2
  Merge2_Simulated249/1 -> Merge2_Simulated272/2
  WC27/1 -> Byte_TwoBusAccess171/4, Byte_TwoBusAccess131/4, Byte_TwoBusAccess91/4, Byte_TwoBusAccess51/4, Byte_TwoBusAccess19/4
  Byte_TwoBusAccess18/1 -> Merge2_Simulated249/2
  Byte_TwoBusAccess131/1 -> Merge2_Simulated264/1
  Byte_TwoBusAccess135/1 -> Merge2_Simulated265/1
  Merge2_Simulated271/1 -> Merge2_Simulated256/2
  Byte_TwoBusAccess136/1 -> Merge2_Simulated261/1
  Byte_TwoBusAccess19/1 -> Merge2_Simulated255/2
  Byte_TwoBusAccess20/1 -> Merge2_Simulated271/2
  Merge2_Simulated254/1 -> Merge2_Simulated263/2
  Merge2_Simulated259/1 -> Merge2_Simulated260/2
  RC33/1 -> Byte_TwoBusAccess25/1, Byte_TwoBusAccess58/1, Byte_TwoBusAccess98/1, Byte_TwoBusAccess178/1, Byte_TwoBusAccess138/1
  Byte_TwoBusAccess107/1 -> Merge2_Simulated276/1
  Byte_TwoBusAccess130/1 -> Merge2_Simulated273/1
  Byte_TwoBusAccess22/1 -> Merge2_Simulated254/2
  Byte_TwoBusAccess133/1 -> Merge2_Simulated257/1
  RC28/1 -> Byte_TwoBusAccess20/1, Byte_TwoBusAccess53/1, Byte_TwoBusAccess93/1, Byte_TwoBusAccess173/1, Byte_TwoBusAccess133/1
  Byte_TwoBusAccess32/1 -> Merge2_Simulated279/2
  WC31/1 -> Byte_TwoBusAccess176/4, Byte_TwoBusAccess136/4, Byte_TwoBusAccess96/4, Byte_TwoBusAccess56/4, Byte_TwoBusAccess23/4
  Byte_TwoBusAccess54/1 -> Merge2_Simulated267/1
  Merge2_Simulated282/1 -> Merge2_Simulated283/2
  Merge2_Simulated334/1 -> Merge2_Simulated51/1
  Merge2_Simulated251/1 -> Merge2_Simulated339/2
  Merge2_Simulated264/1 -> Merge2_Simulated333/2
  Byte_TwoBusAccess175/1 -> Merge2_Simulated334/1
  Merge2_Simulated261/1 -> Merge2_Simulated335/2
  Merge2_Simulated296/1 -> Merge2_Simulated341/2
  Byte_TwoBusAccess187/1 -> Merge2_Simulated338/1
  Merge2_Simulated273/1 -> Merge2_Simulated332/2
  Merge2_Simulated348/1 -> Merge2_Simulated343/2
  Merge2_Simulated289/1 -> Merge2_Simulated345/2
  Byte_TwoBusAccess178/1 -> Merge2_Simulated346/1
  Byte_TwoBusAccess186/1 -> Merge2_Simulated339/1
  RR29/1 -> Byte_TwoBusAccess160/2, Byte_TwoBusAccess161/2, Byte_TwoBusAccess172/2, Byte_TwoBusAccess183/2, Byte_TwoBusAccess194/2, Byte_TwoBusAccess195/2, Byte_TwoBusAccess196/2, Byte_TwoBusAccess197/2, Byte_TwoBusAccess198/2, Byte_TwoBusAccess199/2, Byte_TwoBusAccess162/2, Byte_TwoBusAccess163/2, Byte_TwoBusAccess164/2, Byte_TwoBusAccess165/2, Byte_TwoBusAccess166/2, Byte_TwoBusAccess167/2, Byte_TwoBusAccess169/2, Byte_TwoBusAccess179/2, Byte_TwoBusAccess180/2, Byte_TwoBusAccess181/2, Byte_TwoBusAccess182/2, Byte_TwoBusAccess184/2, Byte_TwoBusAccess185/2, Byte_TwoBusAccess186/2, Byte_TwoBusAccess187/2, Byte_TwoBusAccess170/2, Byte_TwoBusAccess171/2, Byte_TwoBusAccess173/2, Byte_TwoBusAccess174/2, Byte_TwoBusAccess175/2, Byte_TwoBusAccess176/2, Byte_TwoBusAccess177/2, Byte_TwoBusAccess178/2, Byte_TwoBusAccess188/2, Byte_TwoBusAccess189/2, Byte_TwoBusAccess190/2, Byte_TwoBusAccess191/2, Byte_TwoBusAccess193/2, Byte_TwoBusAccess192/2
  Byte_TwoBusAccess192/1 -> Merge2_Simulated342/1
  Merge2_Simulated336/1 -> Merge2_Simulated50/1
  Merge2_Simulated338/1 -> Merge2_Simulated46/1
  Merge2_Simulated265/1 -> Merge2_Simulated334/2
  Merge2_Simulated269/1 -> Merge2_Simulated336/2
  Merge2_Simulated257/1 -> Merge2_Simulated337/2
  Merge2_Simulated337/1 -> Merge2_Simulated49/1
  Merge2_Simulated283/1 -> Merge2_Simulated347/2
  Merge2_Simulated301/1 -> Merge2_Simulated344/2
  Merge2_Simulated333/1 -> Merge2_Simulated48/1
  Byte_TwoBusAccess177/1 -> Merge2_Simulated347/1
  Merge2_Simulated340/1 -> Merge2_Simulated55/1
  Merge2_Simulated345/1 -> Merge2_Simulated59/1
  Merge2_Simulated346/1 -> Merge2_Simulated54/1
  Byte_TwoBusAccess170/1 -> Merge2_Simulated332/1
  Merge2_Simulated277/1 -> Merge2_Simulated338/2
  Byte_TwoBusAccess188/1 -> Merge2_Simulated340/1
  Byte_TwoBusAccess176/1 -> Merge2_Simulated335/1
  Byte_TwoBusAccess189/1 -> Merge2_Simulated341/1
  Byte_TwoBusAccess193/1 -> Merge2_Simulated343/1
  Merge2_Simulated213/1 -> Merge2_Simulated322/2
  Byte_TwoBusAccess162/1 -> Merge2_Simulated312/1
  Byte_TwoBusAccess167/1 -> Merge2_Simulated319/1
  Merge2_Simulated319/1 -> Merge2_Simulated32/1
  Byte_TwoBusAccess179/1 -> Merge2_Simulated324/1
  Byte_TwoBusAccess185/1 -> Merge2_Simulated327/1
  Byte_TwoBusAccess180/1 -> Merge2_Simulated325/1
  Merge2_Simulated241/1 -> Merge2_Simulated324/2
  Merge2_Simulated330/1 -> Merge2_Simulated36/1
  Merge2_Simulated327/1 -> Merge2_Simulated44/1
  Merge2_Simulated325/1 -> Merge2_Simulated38/1
  Merge2_Simulated297/1 -> Merge2_Simulated342/2
  Merge2_Simulated324/1 -> Merge2_Simulated37/1
  Merge2_Simulated329/1 -> Merge2_Simulated39/1
  Merge2_Simulated331/1 -> Merge2_Simulated33/1
  Byte_TwoBusAccess190/1 -> Merge2_Simulated345/1
  Merge2_Simulated335/1 -> Merge2_Simulated52/1
  Merge2_Simulated315/1 -> Merge2_Simulated21/1
  RC07/1 -> Byte_TwoBusAccess7/1, Byte_TwoBusAccess77/1, Byte_TwoBusAccess117/1, Byte_TwoBusAccess197/1, Byte_TwoBusAccess157/1
  Merge2_Simulated342/1 -> Merge2_Simulated61/1
  Merge2_Simulated309/1 -> Merge2_Simulated346/2
  Byte_TwoBusAccess165/1 -> Merge2_Simulated320/1
  Merge2_Simulated201/1 -> Merge2_Simulated314/2
  Merge2_Simulated322/1 -> Merge2_Simulated24/1
  Byte_TwoBusAccess184/1 -> Merge2_Simulated326/1
  Merge2_Simulated341/1 -> Merge2_Simulated58/1
  Merge2_Simulated232/1 -> Merge2_Simulated325/2
  Merge2_Simulated320/1 -> Merge2_Simulated28/1
  Merge2_Simulated205/1 -> Merge2_Simulated320/2
  Byte_TwoBusAccess196/1 -> Merge2_Simulated315/1
  Merge2_Simulated316/1 -> Merge2_Simulated22/1
  Merge2_Simulated317/1 -> Merge2_Simulated20/1
  Byte_TwoBusAccess194/1 -> Merge2_Simulated318/1
  Merge2_Simulated326/1 -> Merge2_Simulated41/1
  Byte_TwoBusAccess195/1 -> Merge2_Simulated317/1
  Merge2_Simulated245/1 -> Merge2_Simulated330/2
  Byte_TwoBusAccess198/1 -> Merge2_Simulated323/1
  Byte_TwoBusAccess197/1 -> Merge2_Simulated316/1
  Byte_TwoBusAccess169/1 -> Merge2_Simulated330/1
  Merge2_Simulated225/1 -> Merge2_Simulated329/2
  Merge2_Simulated314/1 -> Merge2_Simulated29/1
  Byte_TwoBusAccess191/1 -> Merge2_Simulated344/1
  Merge2_Simulated193/1 -> Merge2_Simulated321/2
  Merge2_Simulated237/1 -> Merge2_Simulated328/2
  Byte_TwoBusAccess168/1 -> Merge2_Simulated331/1
  Merge2_Simulated339/1 -> Merge2_Simulated45/1
  Merge2_Simulated332/1 -> Merge2_Simulated47/1
  Byte_TwoBusAccess173/1 -> Merge2_Simulated337/1
  Merge2_Simulated229/1 -> Merge2_Simulated327/2
  Merge2_Simulated318/1 -> Merge2_Simulated17/1
  Byte_TwoBusAccess182/1 -> Merge2_Simulated328/1
  Merge2_Simulated209/1 -> Merge2_Simulated312/2
  Merge2_Simulated347/1 -> Merge2_Simulated53/1
  Merge2_Simulated305/1 -> Merge2_Simulated340/2
  Byte_TwoBusAccess199/1 -> Merge2_Simulated322/1
  Byte_TwoBusAccess181/1 -> Merge2_Simulated329/1
  Byte_TwoBusAccess163/1 -> Merge2_Simulated313/1
  Merge2_Simulated344/1 -> Merge2_Simulated60/1
  Byte_TwoBusAccess171/1 -> Merge2_Simulated333/1
  Merge2_Simulated233/1 -> Merge2_Simulated326/2
  WR29/1 -> Byte_TwoBusAccess193/3, Byte_TwoBusAccess192/3, Byte_TwoBusAccess191/3, Byte_TwoBusAccess190/3, Byte_TwoBusAccess189/3, Byte_TwoBusAccess188/3, Byte_TwoBusAccess178/3, Byte_TwoBusAccess177/3, Byte_TwoBusAccess176/3, Byte_TwoBusAccess175/3, Byte_TwoBusAccess174/3, Byte_TwoBusAccess173/3, Byte_TwoBusAccess171/3, Byte_TwoBusAccess170/3, Byte_TwoBusAccess187/3, Byte_TwoBusAccess186/3, Byte_TwoBusAccess185/3, Byte_TwoBusAccess184/3, Byte_TwoBusAccess182/3, Byte_TwoBusAccess181/3, Byte_TwoBusAccess180/3, Byte_TwoBusAccess179/3, Byte_TwoBusAccess169/3, Byte_TwoBusAccess167/3, Byte_TwoBusAccess166/3, Byte_TwoBusAccess165/3, Byte_TwoBusAccess164/3, Byte_TwoBusAccess163/3, Byte_TwoBusAccess162/3, Byte_TwoBusAccess199/3, Byte_TwoBusAccess198/3, Byte_TwoBusAccess197/3, Byte_TwoBusAccess196/3, Byte_TwoBusAccess195/3, Byte_TwoBusAccess194/3, Byte_TwoBusAccess183/3, Byte_TwoBusAccess172/3, Byte_TwoBusAccess161/3, Byte_TwoBusAccess160/3
  Merge2_Simulated131/1 -> Merge2_Simulated318/2
  Merge2_Simulated197/1 -> Merge2_Simulated319/2
  Merge2_Simulated343/1 -> Merge2_Simulated64/1
  Merge2_Simulated219/1 -> Merge2_Simulated331/2
  Byte_TwoBusAccess164/1 -> Merge2_Simulated321/1
  Byte_TwoBusAccess166/1 -> Merge2_Simulated314/1
  Byte_TwoBusAccess174/1 -> Merge2_Simulated336/1
  Merge2_Simulated200/1 -> Merge2_Simulated313/2
  Merge2_Simulated312/1 -> Merge2_Simulated25/1
  Merge2_Simulated107/1 -> Merge2_Simulated323/2
  Merge2_Simulated328/1 -> Merge2_Simulated40/1
  Merge2_Simulated321/1 -> Merge2_Simulated27/1
  Merge2_Simulated313/1 -> Merge2_Simulated26/1
  OrdNumIn(2B)/1 -> Byte_TwoBusAccess162/5, Byte_TwoBusAccess122/5, Byte_TwoBusAccess82/5, Byte_TwoBusAccess42/5, Byte_TwoBusAccess10/5, Byte_TwoBusAccess163/5, Byte_TwoBusAccess123/5, Byte_TwoBusAccess83/5, Byte_TwoBusAccess43/5, Byte_TwoBusAccess11/5, Byte_TwoBusAccess169/5, Byte_TwoBusAccess129/5, Byte_TwoBusAccess89/5, Byte_TwoBusAccess49/5, Byte_TwoBusAccess17/5, Byte_TwoBusAccess182/5, Byte_TwoBusAccess142/5, Byte_TwoBusAccess102/5, Byte_TwoBusAccess62/5, Byte_TwoBusAccess29/5, Byte_TwoBusAccess184/5, Byte_TwoBusAccess144/5, Byte_TwoBusAccess104/5, Byte_TwoBusAccess64/5, Byte_TwoBusAccess30/5, Byte_TwoBusAccess185/5, Byte_TwoBusAccess145/5, Byte_TwoBusAccess105/5, Byte_TwoBusAccess65/5, Byte_TwoBusAccess31/5, Byte_TwoBusAccess170/5, Byte_TwoBusAccess130/5, Byte_TwoBusAccess90/5, Byte_TwoBusAccess50/5, Byte_TwoBusAccess18/5, Byte_TwoBusAccess175/5, Byte_TwoBusAccess135/5, Byte_TwoBusAccess95/5, Byte_TwoBusAccess55/5, Byte_TwoBusAccess22/5, Byte_TwoBusAccess188/5, Byte_TwoBusAccess148/5, Byte_TwoBusAccess108/5, Byte_TwoBusAccess68/5, Byte_TwoBusAccess34/5, Byte_TwoBusAccess189/5, Byte_TwoBusAccess149/5, Byte_TwoBusAccess109/5, Byte_TwoBusAccess69/5, Byte_TwoBusAccess35/5, Byte_TwoBusAccess190/5, Byte_TwoBusAccess150/5, Byte_TwoBusAccess110/5, Byte_TwoBusAccess70/5, Byte_TwoBusAccess36/5, Byte_TwoBusAccess193/5, Byte_TwoBusAccess224/5, Byte_TwoBusAccess223/5, Byte_TwoBusAccess222/5, Byte_TwoBusAccess221/5, Byte_TwoBusAccess220/5, Byte_TwoBusAccess219/5, Byte_TwoBusAccess218/5, Byte_TwoBusAccess217/5, Byte_TwoBusAccess216/5, Byte_TwoBusAccess215/5, Byte_TwoBusAccess214/5, Byte_TwoBusAccess213/5, Byte_TwoBusAccess212/5, Byte_TwoBusAccess211/5, Byte_TwoBusAccess210/5, Byte_TwoBusAccess209/5, Byte_TwoBusAccess208/5, Byte_TwoBusAccess207/5, Byte_TwoBusAccess206/5, Byte_TwoBusAccess205/5, Byte_TwoBusAccess204/5, Byte_TwoBusAccess203/5, Byte_TwoBusAccess202/5, Byte_TwoBusAccess201/5, Byte_TwoBusAccess200/5, Byte_TwoBusAccess153/5, Byte_TwoBusAccess113/5, Byte_TwoBusAccess73/5, Byte_TwoBusAccess39/5, Byte_TwoBusAccess192/5, Byte_TwoBusAccess152/5, Byte_TwoBusAccess112/5, Byte_TwoBusAccess72/5, Byte_TwoBusAccess38/5, Byte_TwoBusAccess191/5, Byte_TwoBusAccess151/5, Byte_TwoBusAccess111/5, Byte_TwoBusAccess71/5, Byte_TwoBusAccess37/5, Byte_TwoBusAccess178/5, Byte_TwoBusAccess138/5, Byte_TwoBusAccess98/5, Byte_TwoBusAccess58/5, Byte_TwoBusAccess25/5, Byte_TwoBusAccess177/5, Byte_TwoBusAccess137/5, Byte_TwoBusAccess97/5, Byte_TwoBusAccess57/5, Byte_TwoBusAccess24/5, Byte_TwoBusAccess176/5, Byte_TwoBusAccess136/5, Byte_TwoBusAccess96/5, Byte_TwoBusAccess56/5, Byte_TwoBusAccess23/5, Byte_TwoBusAccess174/5, Byte_TwoBusAccess134/5, Byte_TwoBusAccess94/5, Byte_TwoBusAccess54/5, Byte_TwoBusAccess21/5, Byte_TwoBusAccess173/5, Byte_TwoBusAccess133/5, Byte_TwoBusAccess93/5, Byte_TwoBusAccess53/5, Byte_TwoBusAccess20/5, Byte_TwoBusAccess171/5, Byte_TwoBusAccess131/5, Byte_TwoBusAccess91/5, Byte_TwoBusAccess51/5, Byte_TwoBusAccess19/5, Byte_TwoBusAccess187/5, Byte_TwoBusAccess147/5, Byte_TwoBusAccess107/5, Byte_TwoBusAccess67/5, Byte_TwoBusAccess33/5, Byte_TwoBusAccess186/5, Byte_TwoBusAccess146/5, Byte_TwoBusAccess106/5, Byte_TwoBusAccess66/5, Byte_TwoBusAccess32/5, Byte_TwoBusAccess181/5, Byte_TwoBusAccess141/5, Byte_TwoBusAccess101/5, Byte_TwoBusAccess61/5, Byte_TwoBusAccess28/5, Byte_TwoBusAccess180/5, Byte_TwoBusAccess140/5, Byte_TwoBusAccess100/5, Byte_TwoBusAccess60/5, Byte_TwoBusAccess27/5, Byte_TwoBusAccess179/5, Byte_TwoBusAccess139/5, Byte_TwoBusAccess99/5, Byte_TwoBusAccess59/5, Byte_TwoBusAccess26/5, Byte_TwoBusAccess168/5, Byte_TwoBusAccess128/5, Byte_TwoBusAccess88/5, Byte_TwoBusAccess48/5, Byte_TwoBusAccess16/5, Byte_TwoBusAccess167/5, Byte_TwoBusAccess127/5, Byte_TwoBusAccess87/5, Byte_TwoBusAccess47/5, Byte_TwoBusAccess15/5, Byte_TwoBusAccess166/5, Byte_TwoBusAccess126/5, Byte_TwoBusAccess86/5, Byte_TwoBusAccess46/5, Byte_TwoBusAccess14/5, Byte_TwoBusAccess165/5, Byte_TwoBusAccess125/5, Byte_TwoBusAccess85/5, Byte_TwoBusAccess45/5, Byte_TwoBusAccess13/5, Byte_TwoBusAccess164/5, Byte_TwoBusAccess124/5, Byte_TwoBusAccess84/5, Byte_TwoBusAccess44/5, Byte_TwoBusAccess12/5, Byte_TwoBusAccess199/5, Byte_TwoBusAccess159/5, Byte_TwoBusAccess119/5, Byte_TwoBusAccess79/5, Byte_TwoBusAccess9/5, Byte_TwoBusAccess198/5, Byte_TwoBusAccess158/5, Byte_TwoBusAccess118/5, Byte_TwoBusAccess78/5, Byte_TwoBusAccess8/5, Byte_TwoBusAccess197/5, Byte_TwoBusAccess157/5, Byte_TwoBusAccess117/5, Byte_TwoBusAccess77/5, Byte_TwoBusAccess7/5, Byte_TwoBusAccess196/5, Byte_TwoBusAccess156/5, Byte_TwoBusAccess116/5, Byte_TwoBusAccess76/5, Byte_TwoBusAccess6/5, Byte_TwoBusAccess195/5, Byte_TwoBusAccess155/5, Byte_TwoBusAccess115/5, Byte_TwoBusAccess75/5, Byte_TwoBusAccess5/5, Byte_TwoBusAccess194/5, Byte_TwoBusAccess154/5, Byte_TwoBusAccess114/5, Byte_TwoBusAccess74/5, Byte_TwoBusAccess4/5, Byte_TwoBusAccess183/5, Byte_TwoBusAccess143/5, Byte_TwoBusAccess103/5, Byte_TwoBusAccess63/5, Byte_TwoBusAccess3/5, Byte_TwoBusAccess172/5, Byte_TwoBusAccess132/5, Byte_TwoBusAccess92/5, Byte_TwoBusAccess52/5, Byte_TwoBusAccess2/5, Byte_TwoBusAccess161/5, Byte_TwoBusAccess121/5, Byte_TwoBusAccess81/5, Byte_TwoBusAccess41/5, Byte_TwoBusAccess1/5, Byte_TwoBusAccess160/5, Byte_TwoBusAccess249/5, Byte_TwoBusAccess248/5, Byte_TwoBusAccess247/5, Byte_TwoBusAccess246/5, Byte_TwoBusAccess245/5, Byte_TwoBusAccess244/5, Byte_TwoBusAccess243/5, Byte_TwoBusAccess242/5, Byte_TwoBusAccess241/5, Byte_TwoBusAccess240/5, Byte_TwoBusAccess239/5, Byte_TwoBusAccess238/5, Byte_TwoBusAccess237/5, Byte_TwoBusAccess236/5, Byte_TwoBusAccess235/5, Byte_TwoBusAccess234/5, Byte_TwoBusAccess233/5, Byte_TwoBusAccess232/5, Byte_TwoBusAccess231/5, Byte_TwoBusAccess230/5, Byte_TwoBusAccess229/5, Byte_TwoBusAccess228/5, Byte_TwoBusAccess227/5, Byte_TwoBusAccess226/5, Byte_TwoBusAccess225/5, Byte_TwoBusAccess120/5, Byte_TwoBusAccess80/5, Byte_TwoBusAccess40/5, Byte_TwoBusAccess/5
  RR04/1 -> Byte_TwoBusAccess225/2, Byte_TwoBusAccess200/2
  Byte_TwoBusAccess211/1 -> Merge2_Simulated171/1
  Byte_TwoBusAccess200/1 -> Merge2_Simulated141/1
  Merge2_Simulated169/1 -> Merge2_Simulated170/2
  Byte_TwoBusAccess205/1 -> Merge2_Simulated159/1
  Merge2_Simulated143/1 -> Merge2_Simulated144/2
  Byte_TwoBusAccess210/1 -> Merge2_Simulated170/1
  Merge2_Simulated161/1 -> Merge2_Simulated168/2
  WC39/1 -> Byte_TwoBusAccess193/4, Byte_TwoBusAccess224/4, Byte_TwoBusAccess223/4, Byte_TwoBusAccess222/4, Byte_TwoBusAccess221/4, Byte_TwoBusAccess220/4, Byte_TwoBusAccess219/4, Byte_TwoBusAccess218/4, Byte_TwoBusAccess217/4, Byte_TwoBusAccess216/4, Byte_TwoBusAccess215/4, Byte_TwoBusAccess214/4, Byte_TwoBusAccess213/4, Byte_TwoBusAccess212/4, Byte_TwoBusAccess211/4, Byte_TwoBusAccess210/4, Byte_TwoBusAccess209/4, Byte_TwoBusAccess208/4, Byte_TwoBusAccess207/4, Byte_TwoBusAccess206/4, Byte_TwoBusAccess205/4, Byte_TwoBusAccess204/4, Byte_TwoBusAccess203/4, Byte_TwoBusAccess202/4, Byte_TwoBusAccess201/4, Byte_TwoBusAccess200/4, Byte_TwoBusAccess153/4, Byte_TwoBusAccess113/4, Byte_TwoBusAccess73/4, Byte_TwoBusAccess39/4
  Byte_TwoBusAccess207/1 -> Merge2_Simulated161/1
  Byte_TwoBusAccess209/1 -> Merge2_Simulated169/1
  Byte_TwoBusAccess202/1 -> Merge2_Simulated143/1
  Merge2_Simulated293/1 -> Merge2_Simulated141/2
  WR04/1 -> Byte_TwoBusAccess225/3, Byte_TwoBusAccess200/3
  Merge2_Simulated141/1 -> Merge2_Simulated142/2
  Merge2_Simulated168/1 -> Merge2_Simulated169/2
  Byte_TwoBusAccess208/1 -> Merge2_Simulated168/1
  Byte_TwoBusAccess206/1 -> Merge2_Simulated160/1
  Merge2_Simulated144/1 -> Merge2_Simulated158/2
  Byte_TwoBusAccess204/1 -> Merge2_Simulated158/1
  Merge2_Simulated159/1 -> Merge2_Simulated160/2
  Byte_TwoBusAccess203/1 -> Merge2_Simulated144/1
  Merge2_Simulated158/1 -> Merge2_Simulated159/2
  Merge2_Simulated170/1 -> Merge2_Simulated171/2
  Merge2_Simulated142/1 -> Merge2_Simulated143/2
  Merge2_Simulated160/1 -> Merge2_Simulated161/2
  Byte_TwoBusAccess201/1 -> Merge2_Simulated142/1
  Merge2_Simulated136/1 -> Merge2_Simulated137/2
  Byte_TwoBusAccess220/1 -> Merge2_Simulated163/1
  Merge2_Simulated146/1 -> Merge2_Simulated154/2
  Byte_TwoBusAccess216/1 -> Merge2_Simulated154/1
  Byte_TwoBusAccess217/1 -> Merge2_Simulated155/1
  Merge2_Simulated172/1 -> Merge2_Simulated174/2
  Byte_TwoBusAccess213/1 -> Merge2_Simulated137/1
  Byte_TwoBusAccess221/1 -> Merge2_Simulated164/1
  Merge2_Simulated171/1 -> Merge2_Simulated136/2
  Byte_TwoBusAccess214/1 -> Merge2_Simulated145/1
  Byte_TwoBusAccess222/1 -> Merge2_Simulated172/1
  Byte_TwoBusAccess219/1 -> Merge2_Simulated179/1
  Merge2_Simulated179/1 -> Merge2_Simulated163/2
  Merge2_Simulated164/1 -> Merge2_Simulated172/2
  Merge2_Simulated167/1 -> Merge2_Simulated179/2
  Merge2_Simulated155/1 -> Merge2_Simulated167/2
  Byte_TwoBusAccess212/1 -> Merge2_Simulated136/1
  Byte_TwoBusAccess218/1 -> Merge2_Simulated167/1
  Merge2_Simulated145/1 -> Merge2_Simulated146/2
  Byte_TwoBusAccess223/1 -> Merge2_Simulated174/1
  Byte_TwoBusAccess215/1 -> Merge2_Simulated146/1
  Merge2_Simulated154/1 -> Merge2_Simulated155/2
  Merge2_Simulated163/1 -> Merge2_Simulated164/2
  Merge2_Simulated137/1 -> Merge2_Simulated145/2
  Merge2_Simulated174/1 -> Merge2_Simulated348/2
  Byte_TwoBusAccess224/1 -> Merge2_Simulated348/1
  RC39/1 -> Byte_TwoBusAccess39/1, Byte_TwoBusAccess73/1, Byte_TwoBusAccess113/1, Byte_TwoBusAccess153/1, Byte_TwoBusAccess200/1, Byte_TwoBusAccess201/1, Byte_TwoBusAccess202/1, Byte_TwoBusAccess203/1, Byte_TwoBusAccess204/1, Byte_TwoBusAccess205/1, Byte_TwoBusAccess206/1, Byte_TwoBusAccess207/1, Byte_TwoBusAccess208/1, Byte_TwoBusAccess209/1, Byte_TwoBusAccess210/1, Byte_TwoBusAccess211/1, Byte_TwoBusAccess212/1, Byte_TwoBusAccess213/1, Byte_TwoBusAccess214/1, Byte_TwoBusAccess215/1, Byte_TwoBusAccess216/1, Byte_TwoBusAccess217/1, Byte_TwoBusAccess218/1, Byte_TwoBusAccess219/1, Byte_TwoBusAccess220/1, Byte_TwoBusAccess221/1, Byte_TwoBusAccess222/1, Byte_TwoBusAccess223/1, Byte_TwoBusAccess224/1, Byte_TwoBusAccess193/1
  RC08/1 -> Byte_TwoBusAccess8/1, Byte_TwoBusAccess78/1, Byte_TwoBusAccess118/1, Byte_TwoBusAccess198/1, Byte_TwoBusAccess158/1
  RC16/1 -> Byte_TwoBusAccess16/1, Byte_TwoBusAccess48/1, Byte_TwoBusAccess88/1, Byte_TwoBusAccess168/1, Byte_TwoBusAccess128/1
  RC21/1 -> Byte_TwoBusAccess29/1, Byte_TwoBusAccess62/1, Byte_TwoBusAccess102/1, Byte_TwoBusAccess182/1, Byte_TwoBusAccess142/1
  RC03/1 -> Byte_TwoBusAccess3/1, Byte_TwoBusAccess63/1, Byte_TwoBusAccess103/1, Byte_TwoBusAccess183/1, Byte_TwoBusAccess143/1
  RC05/1 -> Byte_TwoBusAccess5/1, Byte_TwoBusAccess75/1, Byte_TwoBusAccess115/1, Byte_TwoBusAccess195/1, Byte_TwoBusAccess155/1
  RC24/1 -> Byte_TwoBusAccess32/1, Byte_TwoBusAccess66/1, Byte_TwoBusAccess106/1, Byte_TwoBusAccess186/1, Byte_TwoBusAccess146/1
  RC31/1 -> Byte_TwoBusAccess23/1, Byte_TwoBusAccess56/1, Byte_TwoBusAccess96/1, Byte_TwoBusAccess176/1, Byte_TwoBusAccess136/1
  RC32/1 -> Byte_TwoBusAccess24/1, Byte_TwoBusAccess57/1, Byte_TwoBusAccess97/1, Byte_TwoBusAccess177/1, Byte_TwoBusAccess137/1
  RC37/1 -> Byte_TwoBusAccess37/1, Byte_TwoBusAccess71/1, Byte_TwoBusAccess111/1, Byte_TwoBusAccess191/1, Byte_TwoBusAccess151/1
  WC32/1 -> Byte_TwoBusAccess177/4, Byte_TwoBusAccess137/4, Byte_TwoBusAccess97/4, Byte_TwoBusAccess57/4, Byte_TwoBusAccess24/4
  WC02/1 -> Byte_TwoBusAccess172/4, Byte_TwoBusAccess132/4, Byte_TwoBusAccess92/4, Byte_TwoBusAccess52/4, Byte_TwoBusAccess2/4
  WC03/1 -> Byte_TwoBusAccess183/4, Byte_TwoBusAccess143/4, Byte_TwoBusAccess103/4, Byte_TwoBusAccess63/4, Byte_TwoBusAccess3/4
  WC04/1 -> Byte_TwoBusAccess194/4, Byte_TwoBusAccess154/4, Byte_TwoBusAccess114/4, Byte_TwoBusAccess74/4, Byte_TwoBusAccess4/4
  WC05/1 -> Byte_TwoBusAccess195/4, Byte_TwoBusAccess155/4, Byte_TwoBusAccess115/4, Byte_TwoBusAccess75/4, Byte_TwoBusAccess5/4
  WC06/1 -> Byte_TwoBusAccess196/4, Byte_TwoBusAccess156/4, Byte_TwoBusAccess116/4, Byte_TwoBusAccess76/4, Byte_TwoBusAccess6/4
  WC07/1 -> Byte_TwoBusAccess197/4, Byte_TwoBusAccess157/4, Byte_TwoBusAccess117/4, Byte_TwoBusAccess77/4, Byte_TwoBusAccess7/4
  WC08/1 -> Byte_TwoBusAccess198/4, Byte_TwoBusAccess158/4, Byte_TwoBusAccess118/4, Byte_TwoBusAccess78/4, Byte_TwoBusAccess8/4
  Merge2_Simulated189/1 -> Merge2_Simulated317/2
  Merge2_Simulated151/1 -> Merge2_Simulated315/2
  Merge2_Simulated135/1 -> Merge2_Simulated316/2
  WC16/1 -> Byte_TwoBusAccess168/4, Byte_TwoBusAccess128/4, Byte_TwoBusAccess88/4, Byte_TwoBusAccess48/4, Byte_TwoBusAccess16/4
  WC24/1 -> Byte_TwoBusAccess186/4, Byte_TwoBusAccess146/4, Byte_TwoBusAccess106/4, Byte_TwoBusAccess66/4, Byte_TwoBusAccess32/4
  WR05/1 -> Byte_TwoBusAccess226/3, Byte_TwoBusAccess201/3
  WR06/1 -> Byte_TwoBusAccess227/3, Byte_TwoBusAccess202/3
  WR07/1 -> Byte_TwoBusAccess228/3, Byte_TwoBusAccess203/3
  WR08/1 -> Byte_TwoBusAccess229/3, Byte_TwoBusAccess204/3
  WR09/1 -> Byte_TwoBusAccess230/3, Byte_TwoBusAccess205/3
  WR10/1 -> Byte_TwoBusAccess231/3, Byte_TwoBusAccess206/3
  WR11/1 -> Byte_TwoBusAccess232/3, Byte_TwoBusAccess207/3
  WR12/1 -> Byte_TwoBusAccess233/3, Byte_TwoBusAccess208/3
  WR13/1 -> Byte_TwoBusAccess234/3, Byte_TwoBusAccess209/3
  WR14/1 -> Byte_TwoBusAccess235/3, Byte_TwoBusAccess210/3
  WR15/1 -> Byte_TwoBusAccess236/3, Byte_TwoBusAccess211/3
  WR16/1 -> Byte_TwoBusAccess237/3, Byte_TwoBusAccess212/3
  WR17/1 -> Byte_TwoBusAccess238/3, Byte_TwoBusAccess213/3
  WR18/1 -> Byte_TwoBusAccess239/3, Byte_TwoBusAccess214/3
  WR19/1 -> Byte_TwoBusAccess240/3, Byte_TwoBusAccess215/3
  WR20/1 -> Byte_TwoBusAccess241/3, Byte_TwoBusAccess216/3
  WR21/1 -> Byte_TwoBusAccess242/3, Byte_TwoBusAccess217/3
  WR22/1 -> Byte_TwoBusAccess243/3, Byte_TwoBusAccess218/3
  WR23/1 -> Byte_TwoBusAccess244/3, Byte_TwoBusAccess219/3
  WR24/1 -> Byte_TwoBusAccess245/3, Byte_TwoBusAccess220/3
  WR25/1 -> Byte_TwoBusAccess246/3, Byte_TwoBusAccess221/3
  WR26/1 -> Byte_TwoBusAccess247/3, Byte_TwoBusAccess222/3
  WR27/1 -> Byte_TwoBusAccess248/3, Byte_TwoBusAccess223/3
  WR28/1 -> Byte_TwoBusAccess249/3, Byte_TwoBusAccess224/3
  RR05/1 -> Byte_TwoBusAccess226/2, Byte_TwoBusAccess201/2
  RR06/1 -> Byte_TwoBusAccess227/2, Byte_TwoBusAccess202/2
  RR07/1 -> Byte_TwoBusAccess228/2, Byte_TwoBusAccess203/2
  RR08/1 -> Byte_TwoBusAccess229/2, Byte_TwoBusAccess204/2
  RR09/1 -> Byte_TwoBusAccess230/2, Byte_TwoBusAccess205/2
  RR10/1 -> Byte_TwoBusAccess231/2, Byte_TwoBusAccess206/2
  RR11/1 -> Byte_TwoBusAccess232/2, Byte_TwoBusAccess207/2
  RR12/1 -> Byte_TwoBusAccess233/2, Byte_TwoBusAccess208/2
  RR13/1 -> Byte_TwoBusAccess234/2, Byte_TwoBusAccess209/2
  RR14/1 -> Byte_TwoBusAccess235/2, Byte_TwoBusAccess210/2
  RR15/1 -> Byte_TwoBusAccess236/2, Byte_TwoBusAccess211/2
  RR16/1 -> Byte_TwoBusAccess237/2, Byte_TwoBusAccess212/2
  RR17/1 -> Byte_TwoBusAccess238/2, Byte_TwoBusAccess213/2
  RR18/1 -> Byte_TwoBusAccess239/2, Byte_TwoBusAccess214/2
  RR19/1 -> Byte_TwoBusAccess240/2, Byte_TwoBusAccess215/2
  RR20/1 -> Byte_TwoBusAccess241/2, Byte_TwoBusAccess216/2
  RR21/1 -> Byte_TwoBusAccess242/2, Byte_TwoBusAccess217/2
  RR22/1 -> Byte_TwoBusAccess243/2, Byte_TwoBusAccess218/2
  RR23/1 -> Byte_TwoBusAccess244/2, Byte_TwoBusAccess219/2
  RR24/1 -> Byte_TwoBusAccess245/2, Byte_TwoBusAccess220/2
  RR25/1 -> Byte_TwoBusAccess246/2, Byte_TwoBusAccess221/2
  RR26/1 -> Byte_TwoBusAccess247/2, Byte_TwoBusAccess222/2
  RR27/1 -> Byte_TwoBusAccess248/2, Byte_TwoBusAccess223/2
  RR28/1 -> Byte_TwoBusAccess249/2, Byte_TwoBusAccess224/2
  Merge2_Simulated112/1 -> Merge2_Simulated4/1
  Merge2_Simulated117/1 -> Merge2_Simulated4/2
  Merge2_Simulated4/1 -> Merge2_Simulated8/2
  Merge2_Simulated100/1 -> Merge2_Simulated8/1
  Merge2_Simulated8/1 -> Merge2_Simulated12/2
  Merge2_Simulated105/1 -> Merge2_Simulated12/1
  Merge2_Simulated12/1 -> Merge2_Simulated17/2
  Merge2_Simulated17/1 -> Merge2_Simulated20/2
  Merge2_Simulated20/1 -> Merge2_Simulated21/2
  Merge2_Simulated21/1 -> Merge2_Simulated22/2
  Merge2_Simulated323/1 -> Merge2_Simulated23/1
  Merge2_Simulated22/1 -> Merge2_Simulated23/2
  Merge2_Simulated23/1 -> Merge2_Simulated24/2
  Merge2_Simulated24/1 -> Merge2_Simulated25/2
  Merge2_Simulated25/1 -> Merge2_Simulated26/2
  Merge2_Simulated26/1 -> Merge2_Simulated27/2
  Merge2_Simulated27/1 -> Merge2_Simulated28/2
  Merge2_Simulated28/1 -> Merge2_Simulated29/2
  Merge2_Simulated29/1 -> Merge2_Simulated32/2
  Merge2_Simulated32/1 -> Merge2_Simulated33/2
  Merge2_Simulated33/1 -> Merge2_Simulated36/2
  Merge2_Simulated36/1 -> Merge2_Simulated37/2
  Merge2_Simulated37/1 -> Merge2_Simulated38/2
  Merge2_Simulated38/1 -> Merge2_Simulated39/2
  Merge2_Simulated39/1 -> Merge2_Simulated40/2
  Merge2_Simulated40/1 -> Merge2_Simulated41/2
  Merge2_Simulated41/1 -> Merge2_Simulated44/2
  Merge2_Simulated44/1 -> Merge2_Simulated45/2
  Merge2_Simulated45/1 -> Merge2_Simulated46/2
  Merge2_Simulated46/1 -> Merge2_Simulated47/2
  Merge2_Simulated47/1 -> Merge2_Simulated48/2
  Merge2_Simulated48/1 -> Merge2_Simulated49/2
  Merge2_Simulated49/1 -> Merge2_Simulated50/2
  Merge2_Simulated50/1 -> Merge2_Simulated51/2
  Merge2_Simulated51/1 -> Merge2_Simulated52/2
  Merge2_Simulated52/1 -> Merge2_Simulated53/2
  Merge2_Simulated53/1 -> Merge2_Simulated54/2
  Merge2_Simulated54/1 -> Merge2_Simulated55/2
  Merge2_Simulated55/1 -> Merge2_Simulated58/2
  Merge2_Simulated58/1 -> Merge2_Simulated59/2
  Merge2_Simulated59/1 -> Merge2_Simulated60/2
  Merge2_Simulated60/1 -> Merge2_Simulated61/2
  Merge2_Simulated61/1 -> Merge2_Simulated64/2
  Merge2_Simulated64/1 -> OrdNumOut(1B)/1
